simulink library "inp"  (R2021b)
settings: Solver=VariableStepAuto  StartTime=0.0  StopTime=10.0  RelTol=1e-3
undefined symbols (not defined in the file): C_TASK_5MS_S, FALSE, KINP_AcoreReadyToSlp_flg_ovrdflg, KINP_AcoreReadyToSlp_flg_ovrdval, KINP_AllowMovThd_OTA_enum_ovrdflg, KINP_AllowMovThd_OTA_enum_ovrdval, KINP_APSAngleTarget_Deg_ovrdflg, KINP_APSAngleTarget_Deg_ovrdval, KINP_APSDecReq_mps2_ovrdflg, KINP_APSDecReq_mps2_ovrdval, KINP_APSDecReqA_flg_ovrdflg, KINP_APSDecReqA_flg_ovrdval, KINP_APSDFLL_cm_ovrdflg, KINP_APSDFLL_cm_ovrdval, KINP_APSDFLR_cm_ovrdflg, KINP_APSDFLR_cm_ovrdval, KINP_APSDRLL_cm_ovrdflg, KINP_APSDRLL_cm_ovrdval, KINP_APSDRLR_cm_ovrdflg, KINP_APSDRLR_cm_ovrdval, KINP_APSExitCondition_enum_ovrdflg, KINP_APSExitCondition_enum_ovrdval, KINP_APSHWVer_enum_ovrdflg, KINP_APSHWVer_enum_ovrdval, KINP_APSProgressPCT_pct_ovrdflg, KINP_APSProgressPCT_pct_ovrdval, KINP_APSPwrReq_enum_ovrdflg, KINP_APSPwrReq_enum_ovrdval, KINP_APSReq_enum_ovrdflg, KINP_APSReq_enum_ovrdval, KINP_APSRQDisplay_enum_ovrdflg, KINP_APSRQDisplay_enum_ovrdval, KINP_APSRqEPASCtrl_flg_ovrdflg, KINP_APSRqEPASCtrl_flg_ovrdval, KINP_APSShiftPosnReq_enum_ovrdval, KINP_APSShiftPosnReq_enum_ovrflg, KINP_APSSpeedCMD_kph_ovrdval, KINP_APSSpeedCMD_kph_ovrflg, KINP_APSStaSystem_enum_ovrdflg, KINP_APSStaSystem_enum_ovrdval, KINP_APSSWVer_enum_ovrdflg, KINP_APSSWVer_enum_ovrdval, KINP_APSVMCReqA_flg_ovrdval, KINP_APSVMCReqA_flg_ovrflg, KINP_APSVRqEPASCtrl_flg_ovrdflg, KINP_APSVRqEPASCtrl_flg_ovrdval, KINP_AuxBattVolmV_mV_ovrdflg, KINP_AuxBattVolmV_mV_ovrdval, KINP_BTConnectSta_enum_ovrdflg, KINP_BTConnectSta_enum_ovrdval, KINP_CAASSta_enum_ovrdflg, KINP_CAASSta_enum_ovrdval, KINP_CAASVMCReqA_flg_ovrdval, KINP_CAASVMCReqA_flg_ovrflg, KINP_CAN1BusOff_flg_ovrdflg, KINP_CAN1BusOff_flg_ovrdval, KINP_CAN2BusOff_flg_ovrdflg, KINP_CAN2BusOff_flg_ovrdval, KINP_CAN3BusOff_flg_ovrdflg, KINP_CAN3BusOff_flg_ovrdval ... (+222)
libraries: FVT_lib x1035, hcu_lib x1
(part 2 of 33)

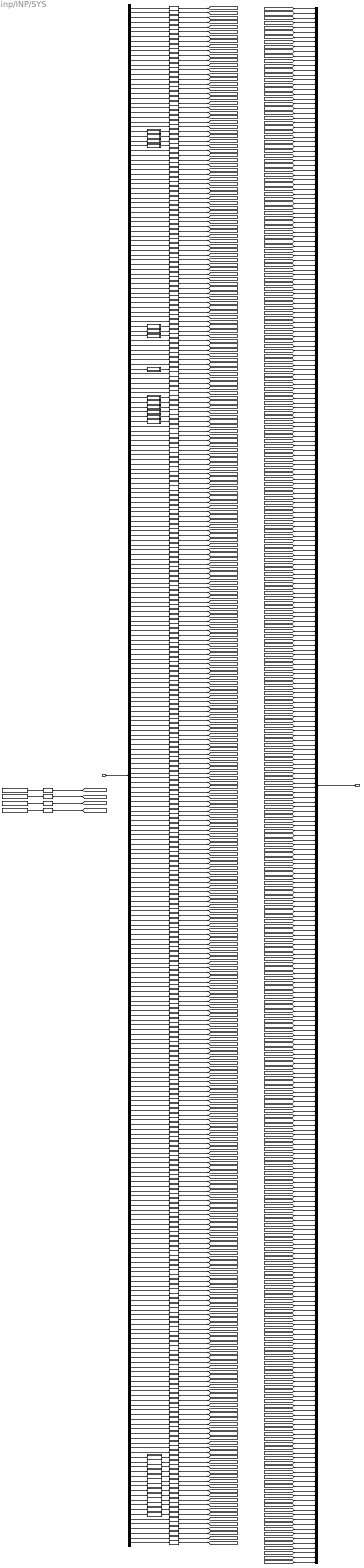
== system inp/INP/SYS ==
  BHAL_SYS_outputs : Inport  OutDataTypeStr=Bus: BHAL_SYS_outputs
  Bus Creator1 : BusCreator  Inputs=328  OutDataTypeStr=Bus: BINP_SYS_outputs  NonVirtualBus=on
  Bus Selector1 : BusSelector  OutputSignals=VHAL_CarMode1_cnt,VHAL_CarModel2_cnt,VHAL_CarModel3_cnt,VHAL_ECU1_cnt,VHAL_ECU2_cnt,VHAL_Major1_cnt,VHAL_Major2_cnt,VHAL_Minor1_cnt,VHAL_Minor2_cnt,VHAL_Patch1_cnt,VHAL_Patch2_cnt,VHAL_Country1_cnt,VHAL_Country2_cnt,VHAL_Variation_cnt,VHAL_Dash1_cnt,VHAL_Change1_cnt,VHAL_Change2_cnt,VHAL_Dash2_cnt,VHAL_SHA1_cnt,VHAL_SHA2_cnt,VHAL_SHA3_cnt,VHAL_SHA4_cnt,VHAL_SHA5_cnt,VHAL_SHA6_cnt,VHAL_SHA7_cnt,VHAL_SHA8_cnt,VHAL_AcoreReadyToSlp_flg,VHAL_PwrReq_OTA_enum,VHAL_AllowMovThd_OTA_enum,VHAL_EvccAplusPwrUpReq_flg,VHAL_DrivetrainSelect_enum,VHAL_ReadFlashCorrect_flg,VHAL_FlashAntitheft_enum,VHAL_RandomnumberY_raw1,VHAL_RandomnumberY_raw2,VHAL_RandomnumberY_raw3,VHAL_RandomnumberY_raw4,VHAL_RandomnumberY_raw5,VHAL_RandomnumberY_raw6,VHAL_RandomnumberY_raw7,VHAL_RandomnumberY_raw8,VHAL_FlashACModeSet123_enum,VHAL_FlashFace_enum,VHAL_FlashFoot_enum,VHAL_FlashFrost_enum,VHAL_FlashFaceM_enum,VHAL_FlashFootM_enum,VHAL_FlashCCUSyncSts_enum,VHAL_FlashACForceOFF_flg,VHAL_FlashsigRecircSt_enum,VHAL_FlashRecAutoFlg_enum,VHAL_FlashAirIntenZone1M_enum,VHAL_Flashfdefog_enum,VHAL_FlashsigSetTempZon1St_C,VHAL_FlashsigSetTempZon2StM_C,VHAL_FlashCountAlarm_enum,VHAL_FlashMFSWTri_flg,VHAL_FlashMirrorFlodPos_flg,VHAL_FlashFuelDoorPos_flg,VHAL_FlashLockSetting_enum,VHAL_FlashMFRDNBrightReq_pct,VHAL_FlashRoomLampMode_enum,VHAL_FlashWiperFixMode_flg,VHAL_FlashIVIPTGUSStaSW_enum,VHAL_AnyNMID_flg,VHAL_CurrentNmState_enum,VHAL_NvmProtectSta_flg,VHAL_AuxBattVolmV_mV,VHAL_Pedal1Ref5V_V,VHAL_Pedal2Ref5V_V,VHAL_EAPS1MINMem_pct,VHAL_EAPS2MINMem_pct,VHAL_FlashHoodSW_flg,VHAL_FlashTailgateSW_flg,VHAL_FlashCTDLockSW_flg,VHAL_FlashTailgateHDSW_flg,VHAL_NetworkReqCalled_flg,VHAL_PmicBootReason_enum,VHAL_WisrBootReason_raw32,VHAL_FlashAPMDoorControlSta_flg,VHAL_AcoreRebootCmd_flg,VHAL_DIDGetDynoMode_flg,VHAL_CAN1BusOff_flg,VHAL_CAN2BusOff_flg,VHAL_CAN3BusOff_flg,VHAL_CAN4BusOff_flg,VHAL_CAN5BusOff_flg,VHAL_CAN6BusOff_flg,VHAL_funAuto_flg,VHAL_DiagDRLOFF_flg,VHAL_DiagFMHT_s,VHAL_DiagFLTC_mA,VHAL_DiagFRTC_mA,VHAL_DiagRLTC_mA,VHAL_DiagRRTC_mA,VHAL_USSConfig_raw8,VHAL_TireSize_raw8,VHAL_APSFunConfig_raw8,VHAL_FlashfUnlockSingle_flg,VHAL_FlashRegenMode_enum,VHAL_FlashAmbFunEN_enum,VHAL_FlashAmbWelEN_enum,VHAL_FlashAmbDimEN_enum,VHAL_FlashAmbLinkDriSta_enum,VHAL_FlashAmbPwrWarnEN_enum,VHAL_FlashAmbODAEN_enum,VHAL_FlashAmbColorSta1_enum,VHAL_FlashAmbColorSta2_enum,VHAL_FlashAmbColorSta3_enum,VHAL_FlashAmbColorSta4_enum,VHAL_FlashAmbColorSta5_enum,VHAL_FlashAmbColorSta7_enum,VHAL_FlashAmbBrightnessSta1_enum,VHAL_FlashAmbBrightnessSta2_enum,VHAL_FlashAmbBrightnessSta3_enum,VHAL_FlashAmbBrightnessSta4_enum,VHAL_FlashAmbBrightnessSta5_enum,VHAL_FlashAmbBrightnessSta7_enum,VHAL_FlashTurnSwTSet123_enum,VHAL_FlashTurnSwTSet457_enum,VHAL_FlashAirIntZ3Sta_enum,VHAL_FlashREVentModeSta_enum,VHAL_FlashLEVentModeSta_enum,VHAL_FlashLEVentZSta_enum,VHAL_FlashCLEVentZSta_enum,VHAL_FlashREVentZSta_enum,VHAL_FlashCREVentZSta_enum,VHAL_FlashLVentEN_enum,VHAL_FlashLEVentYSta_enum,VHAL_FlashCLVentEN_enum,VHAL_FlashCLEVentYSta_enum,VHAL_FlashRVentEN_enum,VHAL_FlashREVentYSta_enum,VHAL_FlashCRVentEN_enum,VHAL_FlashCREVentYSta_enum,VHAL_FlashFGSAirIntSta_enum,VHAL_FlashFGSChSta_enum,VHAL_FlashFGSIONSWSta_enum,VHAL_FlashWalkOutLkEN_enum,VHAL_FlashWalkInUnLkEN_enum,VHAL_FlashFollowMeENFun_enum,VHAL_ResetPedalZeroPosReq_enum,VHAL_FlashPTGUserHeight1_cnt,VHAL_FlashPTGUserHeight2_cnt,VHAL_FlashPTGUserHeight3_cnt,VHAL_FlashPTGUserHeight4_cnt,VHAL_FlashPTGUserHeight5_cnt,VHAL_FlashPTGUserHeight7_cnt,VHAL_FlashPTGOpenHeight12_enum,VHAL_FlashPTGOpenHeight34_enum,VHAL_FlashPTGOpenHeight57_enum,VHAL_FlashACCLevelSta12_enum,VHAL_FlashACCLevelSta34_enum,VHAL_FlashACCLevelSta57_enum,VHAL_AutoWipHSpdEN_flg,VHAL_WipRLSCmdHoldEN_flg,VHAL_WipRLSCmdHoldTime_s,VHAL_WipRLSCmdCutEN_flg,VHAL_WipRLSCmdCutTime_s,VHAL_FlashAutoLock_enum,VHAL_FlashAutoUnlock_enum,VHAL_ECUGen1_cnt,VHAL_ECUGen2_cnt,VHAL_FlashMILDIST_km,VHAL_FlashWARMUPS_cnt,VHAL_FlashCLRDIST_km,VHAL_FlashMILTIME_min,VHAL_FlashCLRTIME_min,VHAL_FlashNUMPSATRIPSFLTMEMCLR_cnt,VHAL_FlashODOMETER_km,VHAL_FlashPSAR_sec,VHAL_FlashPSAL_sec,VHAL_FlashIPSAR_sec,VHAL_FlashIPSAL_sec,VHAL_FlashCPSAR_sec,VHAL_FlashCPSAL_sec,VHAL_FlashHVBNAH_Ahr,VHAL_FlashHVBNE_kWh,VHAL_FlashIGNCNTR_cnt,VHAL_FlashTNBCPSAR_Ahr,VHAL_FlashTNBCPSAL_Ahr,VHAL_FlashTNECPSAR_kWh,VHAL_FlashTNECPSAL_kWh,VHAL_FlashTEBPSAR_kWh,VHAL_FlashTEBPSAL_kWh,VHAL_FlashTGEOVCR_kWh,VHAL_FlashTGEOVCL_kWh,VHAL_FlashGECHGOVCDCR_kWh,VHAL_FlashGECHGOVCDCL_kWh,VHAL_FlashGECHGOVCACR_kWh,VHAL_FlashGECHGOVCACL_kWh,VHAL_FlashRESSV2XENNONPSAR_kWh,VHAL_FlashRESSV2XENNONPSAL_kWh,VHAL_FlashPKERNumerator_kphsqr,VHAL_FlashPKELNumerator_kphsqr,VHAL_FlashResetCDEODTR_km,VHAL_FlashAvgBattTempPSAR_C,VHAL_FlashAvgBattTempPSAL_C,VHAL_FlashAvgBattTempOVCR_C,VHAL_FlashAvgBattTempOVCL_C,VHAL_FlashAvgBattTempOFFR_C,VHAL_FlashAvgBattTempOFFL_C,VHAL_FlashQTYPSATRIPSR_cnt,VHAL_FlashQTYPSATRIPSL_cnt,VHAL_FlashRESSCNTDODRNGR_cnt,VHAL_FlashRESSCNTDODRNGL_cnt,VHAL_FlashETMATOER_kWh,VHAL_FlashETMATOEL_kWh,VHAL_FlashETMBTOER_kWh,VHAL_FlashETMBTOEL_kWh,VHAL_FlashRESSTIMESOCPSARNGR_s,VHAL_FlashRESSTIMESOCPSARNGL_s,VHAL_FlashRESSTIMESOCCHGRNGR_s,VHAL_FlashRESSTIMESOCCHGRNGL_s,VHAL_FlashRESSTIMESOCOFFRNGR_s,VHAL_FlashRESSTIMESOCOFFRNGL_s,VHAL_FlashMAXBATTEMPL_C,VHAL_FlashMINBATTEMPL_C,VHAL_FlashAVGBATTEMPL_sec,VHAL_FlashAVGBATTEMPL_C,VHAL_FlashBattTempPSAR_sec,VHAL_FlashBattTempPSAL_sec,VHAL_FlashOVCR_sec,VHAL_FlashOVCL_sec,VHAL_FlashOFFR_sec,VHAL_FlashOFFL_sec,VHAL_VinCode_cnt,VHAL_FlashHMIKey1Func_enum,VHAL_FlashHMIKey2Func_enum,VHAL_FlashHMIKey3Func_enum,VHAL_FlashHMIKey4Func_enum,VHAL_FlashHMIKey5Func_enum,VHAL_FlashHMIKey6Func_enum,VHAL_FlashHMIKey7Func_enum,VHAL_FlashHMIKey8Func_enum,VHAL_FlashAutoWipHSpdEN_flg,VHAL_PmicBootPath_raw32,VHAL_FlashTPMModelVersion_raw,VHAL_FlashTPMModelVersionChkSum_raw,VHAL_FlashDIDModelVersion_raw,VHAL_FlashDIDModelVersionChkSum_raw,VHAL_FlashAirIntenZone1MSet2_enum,VHAL_FlashAirIntenZone1MSet3_enum,VHAL_FlashAirIntenZone1MSet4_enum,VHAL_FlashAirIntenZone1MSet5_enum,VHAL_FlashAirIntenZone1MSet7_enum,VHAL_FlashAirIntenZone3MSet2_enum,VHAL_FlashAirIntenZone3MSet3_enum,VHAL_FlashAirIntenZone3MSet4_enum,VHAL_FlashAirIntenZone3MSet5_enum,VHAL_FlashAirIntenZone3MSet7_enum,VHAL_FlashFGSChStaSet457_enum,VHAL_FlashFGSAirIntStaSet457_enum,VHAL_FlashLEVentModeStaSet457_enum,VHAL_FlashREVentModeStaSet457_enum,VHAL_FlashLEVentZStaSet2_enum,VHAL_FlashLEVentZStaSet3_enum,VHAL_FlashLEVentZStaSet4_enum,VHAL_FlashLEVentZStaSet5_enum,VHAL_FlashLEVentZStaSet7_enum,VHAL_FlashCLEVentZStaSet2_enum,VHAL_FlashCLEVentZStaSet3_enum,VHAL_FlashCLEVentZStaSet4_enum,VHAL_FlashCLEVentZStaSet5_enum,VHAL_FlashCLEVentZStaSet7_enum,VHAL_FlashREVentZStaSet2_enum,VHAL_FlashREVentZStaSet3_enum,VHAL_FlashREVentZStaSet4_enum,VHAL_FlashREVentZStaSet5_enum,VHAL_FlashREVentZStaSet7_enum,VHAL_FlashCREVentZStaSet2_enum,VHAL_FlashCREVentZStaSet3_enum,VHAL_FlashCREVentZStaSet4_enum,VHAL_FlashCREVentZStaSet5_enum,VHAL_FlashCREVentZStaSet7_enum,VHAL_FlashLEVentYStaSet2_enum,VHAL_FlashLEVentYStaSet3_enum,VHAL_FlashLEVentYStaSet4_enum,VHAL_FlashLEVentYStaSet5_enum,VHAL_FlashLEVentYStaSet7_enum,VHAL_FlashCLEVentYStaSet2_enum,VHAL_FlashCLEVentYStaSet3_enum,VHAL_FlashCLEVentYStaSet4_enum,VHAL_FlashCLEVentYStaSet5_enum,VHAL_FlashCLEVentYStaSet7_enum,VHAL_FlashREVentYStaSet2_enum,VHAL_FlashREVentYStaSet3_enum,VHAL_FlashREVentYStaSet4_enum,VHAL_FlashREVentYStaSet5_enum,VHAL_FlashREVentYStaSet7_enum,VHAL_FlashCREVentYStaSet2_enum,VHAL_FlashCREVentYStaSet3_enum,VHAL_FlashCREVentYStaSet4_enum,VHAL_FlashCREVentYStaSet5_enum,VHAL_FlashCREVentYStaSet7_enum,VHAL_FlashACModeSet457_enum,VHAL_FlashSettempZon1Set2_enum,VHAL_FlashSettempZon1Set3_enum,VHAL_FlashSettempZon1Set4_enum,VHAL_FlashSettempZon1Set5_enum,VHAL_FlashSettempZon1Set7_enum,VHAL_FlashJugKeepUnLZone_flg,VHAL_DrivingMode_cnt,VHAL_ModelYear_cnt,VHAL_FlashCLWinLockDrSta_enum,VHAL_CbnPreACEnaReq_enum,VHAL_PowerOffTSet_cnt,VHAL_ReOutsideMirror_enum,VHAL_ReDoorLock_enum,VHAL_RePwrReqTbox_enum,VHAL_ReRadio_flg,VHAL_RemoteACTemp_C,VHAL_RemoteAutoReq_flg,VHAL_TBOXRemotePW_enum,VHAL_FDCConnDrvWdwCtrlCmd_pct,VHAL_FDCConnPasWdwCtrlCmd_pct,VHAL_FDCConnRLDWdwCtrlCmd_pct,VHAL_FDCConnRRDWdwCtrlCmd_pct,VHAL_CAN1BusError_flg,VHAL_CAN2BusError_flg,VHAL_CAN3BusError_flg,VHAL_CAN4BusError_flg,VHAL_CAN5BusError_flg,VHAL_CAN6BusError_flg
  Constant : Constant  Value=KINP_NewNMSpec_flg
  Constant1 : Constant  Value=KINP_VehicleType_enum
  Constant2 : Constant  Value=KINP_SWCType_enum
  Constant3 : Constant  Value=KINP_SOCDisUsed_flg
  Data Type Conversion{,4,6,12..16,19..27,36,54,57..58,78,81,89,102,112,137..139,147,238,305,314,316,322..327} (40 alike) : DataTypeConversion  OutDataTypeStr=boolean
  Data Type Conversion{1..3,5,17,33..35,37..53,55..56,59..77,79..80,82..88,90..101,103..111,113..122,129..136,140..141,145..146,148,192..209,229..237,240..243,245..304,306..309,311,313,317..321} (201 alike) : DataTypeConversion  OutDataTypeStr=uint8
  Data Type Conversion{8..11,28..32,149..150,154,161..162,164..177,180..186,191,210..212,219..221,310,315} (44 alike) : DataTypeConversion  OutDataTypeStr=single
  Data Type Conversion{7,123..128,151..153,163,189..190,312} (14 alike) : DataTypeConversion  OutDataTypeStr=uint16
  Data Type Conversion{142..144,244} (4 alike) : DataTypeConversion
  Data Type Conversion{18,155..160,178..179,187..188,213..218,222..228,239} (25 alike) : DataTypeConversion  OutDataTypeStr=uint32
  Subsystem : Subsystem
  Subsystem1 : Subsystem
  Subsystem10 : Subsystem
  Subsystem11 : Subsystem
  Subsystem12 : Subsystem
  Subsystem13 : Subsystem
  Subsystem14 : Subsystem
  Subsystem15 : Subsystem
  Subsystem16 : Subsystem
  Subsystem17 : Subsystem
  Subsystem18 : Subsystem
  Subsystem19 : Subsystem
  Subsystem2 : Subsystem
  Subsystem20 : Subsystem
  Subsystem21 : Subsystem
  Subsystem22 : Subsystem
  Subsystem23 : Subsystem
  Subsystem24 : Subsystem
  Subsystem25 : Subsystem
  Subsystem26 : Subsystem
  Subsystem3 : Subsystem
  Subsystem4 : Subsystem
  Subsystem5 : Subsystem
  Subsystem6 : Subsystem
  Subsystem7 : Subsystem
  Subsystem8 : Subsystem
  Subsystem9 : Subsystem
  BINP_SYS_outputs : Outport  OutDataTypeStr=Bus: BINP_SYS_outputs
  wires:
  [VINP_Country2_cnt] -> Bus Creator1/13
  [VINP_FlashAirIntenZone1M_enum] -> Bus Creator1/52
  [VINP_FlashFrost_enum] -> Bus Creator1/45
  Bus Selector1/43 -> Data Type Conversion96/1  "<VHAL_FlashFace_enum>"
  [VINP_FlashCCUSyncSts_enum] -> Bus Creator1/48
  [VINP_EvccAplusPwrUpReq_flg] -> Bus Creator1/30
  Data Type Conversion110/1 -> [VINP_Minor2_cnt]  "VINP_Minor2_cnt"
  Bus Selector1/53 -> Data Type Conversion107/1  "<VHAL_Flashfdefog_enum>"
  [VINP_FlashRecAutoFlg_enum] -> Bus Creator1/51
  Bus Selector1/16 -> Data Type Conversion66/1  "<VHAL_Change1_cnt>"
  [VINP_RandomnumberY_raw1] -> Bus Creator1/34
  Data Type Conversion97/1 -> [VINP_FlashFoot_enum]  "VINP_FlashFoot_enum"
  Bus Selector1/44 -> Data Type Conversion97/1  "<VHAL_FlashFoot_enum>"
  [VINP_FlashFoot_enum] -> Bus Creator1/44
  [VINP_FlashFootM_enum] -> Bus Creator1/47
  Data Type Conversion72/1 -> [VINP_SHA3_cnt]  "VINP_SHA3_cnt"
  [VINP_FlashsigRecircSt_enum] -> Bus Creator1/50
  Data Type Conversion60/1 -> [VINP_CarModel2_cnt]  "VINP_CarModel2_cnt"
  Data Type Conversion100/1 -> [VINP_FlashFootM_enum]  "VINP_FlashFootM_enum"
  Bus Selector1/3 -> Data Type Conversion71/1  "<VHAL_CarModel3_cnt>"
  Data Type Conversion104/1 -> [VINP_Major1_cnt]  "VINP_Major1_cnt"
  [VINP_FlashFaceM_enum] -> Bus Creator1/46
  [VINP_Dash1_cnt] -> Bus Creator1/15
  Bus Selector1/45 -> Data Type Conversion98/1  "<VHAL_FlashFrost_enum>"
  [VINP_FlashACModeMem_enum] -> Bus Creator1/42
  Data Type Conversion108/1 -> [VINP_Major2_cnt]  "VINP_Major2_cnt"
  [VINP_FlashFace_enum] -> Bus Creator1/43
  Bus Selector1/8 -> Data Type Conversion109/1  "<VHAL_Minor1_cnt>"
  [VINP_CarModel1_cnt] -> Bus Creator1/1
  Data Type Conversion82/1 -> [VINP_ECU1_cnt]  "VINP_ECU1_cnt"
  Bus Selector1/47 -> Data Type Conversion100/1  "<VHAL_FlashFootM_enum>"
  Data Type Conversion73/1 -> [VINP_SHA4_cnt]  "VINP_SHA4_cnt"
  Bus Selector1/34 -> Data Type Conversion85/1  "<VHAL_RandomnumberY_raw1>"
  Data Type Conversion84/1 -> [VINP_DrivetrainSelect_enum]  "VINP_DrivetrainSelect_enum"
  Bus Selector1/30 -> Subsystem6/1(In1)  "<VHAL_EvccAplusPwrUpReq_flg>"
  Data Type Conversion101/1 -> [VINP_FlashCCUSyncSts_enum]  "VINP_FlashCCUSyncSts_enum"
  [VINP_DrivetrainSelect_enum] -> Bus Creator1/31
  Data Type Conversion80/1 -> [VINP_AllowMovThd_OTA_enum]  "VINP_AllowMovThd_OTA_enum"
  Bus Selector1/49 -> Data Type Conversion102/1  "<VHAL_FlashACForceOFF_flg>"
  Bus Selector1/38 -> Data Type Conversion90/1  "<VHAL_RandomnumberY_raw5>"
  Bus Selector1/10 -> Data Type Conversion111/1  "<VHAL_Patch1_cnt>"
  Data Type Conversion88/1 -> [VINP_RandomnumberY_raw4]  "VINP_RandomnumberY_raw4"
  [VINP_Flashfdefog_enum] -> Bus Creator1/53
  Bus Selector1/42 -> Data Type Conversion95/1  "<VHAL_FlashACModeSet123_enum>"
  Bus Selector1/37 -> Data Type Conversion88/1  "<VHAL_RandomnumberY_raw4>"
  Bus Selector1/36 -> Data Type Conversion87/1  "<VHAL_RandomnumberY_raw3>"
  Bus Selector1/48 -> Data Type Conversion101/1  "<VHAL_FlashCCUSyncSts_enum>"
  Data Type Conversion102/1 -> [VINP_FlashACForceOFF_flg]  "VINP_FlashACForceOFF_flg"
  [VINP_Change2_cnt] -> Bus Creator1/17
  Bus Selector1/29 -> Subsystem5/1(In1)  "<VHAL_AllowMovThd_OTA_enum>"
  Data Type Conversion63/1 -> [VINP_Country2_cnt]  "VINP_Country2_cnt"
  Data Type Conversion107/1 -> [VINP_Flashfdefog_enum]  "VINP_Flashfdefog_enum"
  Data Type Conversion96/1 -> [VINP_FlashFace_enum]  "VINP_FlashFace_enum"
  [VINP_RandomnumberY_raw2] -> Bus Creator1/35
  [VINP_RandomnumberY_raw6] -> Bus Creator1/39
  [VINP_RandomnumberY_raw4] -> Bus Creator1/37
  [VINP_ECU1_cnt] -> Bus Creator1/4
  Bus Selector1/2 -> Data Type Conversion60/1  "<VHAL_CarModel2_cnt>"
  Data Type Conversion105/1 -> [VINP_FlashRecAutoFlg_enum]  "VINP_FlashRecAutoFlg_enum"
  Data Type Conversion103/1 -> [VINP_FlashsigRecircSt_enum]  "VINP_FlashsigRecircSt_enum"
  Bus Selector1/22 -> Data Type Conversion73/1  "<VHAL_SHA4_cnt>"
  Bus Selector1/46 -> Data Type Conversion99/1  "<VHAL_FlashFaceM_enum>"
  Bus Selector1/50 -> Data Type Conversion103/1  "<VHAL_FlashsigRecircSt_enum>"
  Data Type Conversion98/1 -> [VINP_FlashFrost_enum]  "VINP_FlashFrost_enum"
  [VINP_RandomnumberY_raw5] -> Bus Creator1/38
  [VINP_SHA3_cnt] -> Bus Creator1/21
  Bus Selector1/40 -> Data Type Conversion92/1  "<VHAL_RandomnumberY_raw7>"
  Data Type Conversion86/1 -> [VINP_RandomnumberY_raw2]  "VINP_RandomnumberY_raw2"
  Data Type Conversion111/1 -> [VINP_Patch1_cnt]  "VINP_Patch1_cnt"
  Bus Selector1/35 -> Data Type Conversion86/1  "<VHAL_RandomnumberY_raw2>"
  [VINP_SHA6_cnt] -> Bus Creator1/24
  [VINP_Major1_cnt] -> Bus Creator1/6
  [VINP_RandomnumberY_raw7] -> Bus Creator1/40
  [VINP_RandomnumberY_raw8] -> Bus Creator1/41
  Bus Selector1/15 -> Data Type Conversion65/1  "<VHAL_Dash1_cnt>"
  Data Type Conversion92/1 -> [VINP_RandomnumberY_raw7]  "VINP_RandomnumberY_raw7"
  Data Type Conversion99/1 -> [VINP_FlashFaceM_enum]  "VINP_FlashFaceM_enum"
  Data Type Conversion85/1 -> [VINP_RandomnumberY_raw1]  "VINP_RandomnumberY_raw1"
  Bus Selector1/52 -> Data Type Conversion106/1  "<VHAL_FlashAirIntenZone1M_enum>"
  Data Type Conversion90/1 -> [VINP_RandomnumberY_raw5]  "VINP_RandomnumberY_raw5"
  Data Type Conversion91/1 -> [VINP_RandomnumberY_raw6]  "VINP_RandomnumberY_raw6"
  Data Type Conversion65/1 -> [VINP_Dash1_cnt]  "VINP_Dash1_cnt"
  [VINP_FlashAntitheft_enum] -> Bus Creator1/33
  Data Type Conversion87/1 -> [VINP_RandomnumberY_raw3]  "VINP_RandomnumberY_raw3"
  Bus Selector1/39 -> Data Type Conversion91/1  "<VHAL_RandomnumberY_raw6>"
  [VINP_Dash2_cnt] -> Bus Creator1/18
  Bus Selector1/19 -> Data Type Conversion69/1  "<VHAL_SHA1_cnt>"
  Bus Selector1/41 -> Data Type Conversion94/1  "<VHAL_RandomnumberY_raw8>"
  Data Type Conversion71/1 -> [VINP_CarModel3_cnt]  "VINP_CarModel3_cnt"
  [VINP_SHA4_cnt] -> Bus Creator1/22
  Data Type Conversion76/1 -> [VINP_SHA7_cnt]  "VINP_SHA7_cnt"
  [VINP_AllowMovThd_OTA_enum] -> Bus Creator1/29
  [VINP_ReadFlashCorrect_flg] -> Bus Creator1/32
  Data Type Conversion78/1 -> [VINP_AcoreReadyToSlp_flg]  "VINP_AcoreReadyToSlp_flg"
  Data Type Conversion94/1 -> [VINP_RandomnumberY_raw8]  "VINP_RandomnumberY_raw8"
  Data Type Conversion67/1 -> [VINP_Change2_cnt]  "VINP_Change2_cnt"
  [VINP_CarModel3_cnt] -> Bus Creator1/3
  [VINP_Variation_cnt] -> Bus Creator1/14
  [VINP_SHA2_cnt] -> Bus Creator1/20
  [VINP_FlashACForceOFF_flg] -> Bus Creator1/49
  Bus Selector1/12 -> Data Type Conversion62/1  "<VHAL_Country1_cnt>"
  Bus Selector1/51 -> Data Type Conversion105/1  "<VHAL_FlashRecAutoFlg_enum>"
  Data Type Conversion69/1 -> [VINP_SHA1_cnt]  "VINP_SHA1_cnt"
  [VINP_AcoreReadyToSlp_flg] -> Bus Creator1/27
  [VINP_PwrReq_OTA_enum] -> Bus Creator1/28
  Subsystem4/1(Out1) -> Data Type Conversion79/1
  [VINP_SHA5_cnt] -> Bus Creator1/23
  [VINP_Patch2_cnt] -> Bus Creator1/11
  [VINP_Patch1_cnt] -> Bus Creator1/10
  Data Type Conversion68/1 -> [VINP_Dash2_cnt]  "VINP_Dash2_cnt"
  Subsystem6/1(Out1) -> Data Type Conversion89/1
  Bus Selector1/33 -> Data Type Conversion83/1  "<VHAL_FlashAntitheft_enum>"
  [VINP_Minor2_cnt] -> Bus Creator1/9
  [VINP_SHA7_cnt] -> Bus Creator1/25
  [VINP_Minor1_cnt] -> Bus Creator1/8
  Data Type Conversion95/1 -> [VINP_FlashACModeMem_enum]  "VINP_FlashACModeMem_enum"
  [VINP_CarModel2_cnt] -> Bus Creator1/2
  Data Type Conversion77/1 -> [VINP_SHA8_cnt]  "VINP_SHA8_cnt"
  Data Type Conversion106/1 -> [VINP_FlashAirIntenZone1M_enum]  "VINP_FlashAirIntenZone1M_enum"
  Data Type Conversion66/1 -> [VINP_Change1_cnt]  "VINP_Change1_cnt"
  [VINP_SHA1_cnt] -> Bus Creator1/19
  Data Type Conversion81/1 -> [VINP_ReadFlashCorrect_flg]  "VINP_ReadFlashCorrect_flg"
  [VINP_Country1_cnt] -> Bus Creator1/12
  Bus Selector1/17 -> Data Type Conversion67/1  "<VHAL_Change2_cnt>"
  Data Type Conversion83/1 -> [VINP_FlashAntitheft_enum]  "VINP_FlashAntitheft_enum"
  Data Type Conversion75/1 -> [VINP_SHA6_cnt]  "VINP_SHA6_cnt"
  Data Type Conversion74/1 -> [VINP_SHA5_cnt]  "VINP_SHA5_cnt"
  Data Type Conversion93/1 -> [VINP_ECU2_cnt]  "VINP_ECU2_cnt"
  [VINP_RandomnumberY_raw3] -> Bus Creator1/36
  Data Type Conversion70/1 -> [VINP_SHA2_cnt]  "VINP_SHA2_cnt"
  Bus Selector1/21 -> Data Type Conversion72/1  "<VHAL_SHA3_cnt>"
  Data Type Conversion62/1 -> [VINP_Country1_cnt]  "VINP_Country1_cnt"
  [VINP_ECU2_cnt] -> Bus Creator1/5
  Bus Selector1/31 -> Data Type Conversion84/1  "<VHAL_DrivetrainSelect_enum>"
  Data Type Conversion64/1 -> [VINP_Variation_cnt]  "VINP_Variation_cnt"
  Data Type Conversion61/1 -> [VINP_Patch2_cnt]  "VINP_Patch2_cnt"
  Bus Selector1/18 -> Data Type Conversion68/1  "<VHAL_Dash2_cnt>"
  Bus Selector1/28 -> Subsystem4/1(In1)  "<VHAL_PwrReq_OTA_enum>"
  Bus Selector1/24 -> Data Type Conversion75/1  "<VHAL_SHA6_cnt>"
  Bus Selector1/27 -> Subsystem7/1(In1)  "<VHAL_AcoreReadyToSlp_flg>"
  [VINP_SHA8_cnt] -> Bus Creator1/26
  Bus Selector1/20 -> Data Type Conversion70/1  "<VHAL_SHA2_cnt>"
  Subsystem5/1(Out1) -> Data Type Conversion80/1
  Bus Selector1/25 -> Data Type Conversion76/1  "<VHAL_SHA7_cnt>"
  [VINP_Major2_cnt] -> Bus Creator1/7
  Bus Selector1/32 -> Data Type Conversion81/1  "<VHAL_ReadFlashCorrect_flg>"
  Data Type Conversion59/1 -> [VINP_CarModel1_cnt]  "VINP_CarModel1_cnt"
  Bus Selector1/23 -> Data Type Conversion74/1  "<VHAL_SHA5_cnt>"
  Bus Selector1/14 -> Data Type Conversion64/1  "<VHAL_Variation_cnt>"
  [VINP_Change1_cnt] -> Bus Creator1/16
  Subsystem7/1(Out1) -> Data Type Conversion78/1
  Bus Selector1/13 -> Data Type Conversion63/1  "<VHAL_Country2_cnt>"
  Bus Selector1/4 -> Data Type Conversion82/1  "<VHAL_ECU1_cnt>"
  Data Type Conversion79/1 -> [VINP_PwrReq_OTA_enum]  "VINP_PwrReq_OTA_enum"
  Bus Selector1/7 -> Data Type Conversion108/1  "<VHAL_Major2_cnt>"
  Bus Selector1/9 -> Data Type Conversion110/1  "<VHAL_Minor2_cnt>"
  Bus Selector1/5 -> Data Type Conversion93/1  "<VHAL_ECU2_cnt>"
  Data Type Conversion89/1 -> [VINP_EvccAplusPwrUpReq_flg]  "VINP_EvccAplusPwrUpReq_flg"
  Bus Selector1/1 -> Data Type Conversion59/1  "<VHAL_CarMode1_cnt>"
  Bus Selector1/6 -> Data Type Conversion104/1  "<VHAL_Major1_cnt>"
  Data Type Conversion109/1 -> [VINP_Minor1_cnt]  "VINP_Minor1_cnt"
  BHAL_SYS_outputs/1 -> Bus Selector1/1
  Bus Creator1/1 -> BINP_SYS_outputs/1
  Bus Selector1/11 -> Data Type Conversion61/1  "<VHAL_Patch2_cnt>"
  Bus Selector1/26 -> Data Type Conversion77/1  "<VHAL_SHA8_cnt>"
  Data Type Conversion112/1 -> [VINP_AnyNMID_flg]  "VINP_AnyNMID_flg"
  Data Type Conversion113/1 -> [VINP_CurrentNmState_enum]  "VINP_CurrentNmState_enum"
  Bus Selector1/65 -> Data Type Conversion112/1  "<VHAL_AnyNMID_flg>"
  Bus Selector1/66 -> Data Type Conversion113/1  "<VHAL_CurrentNmState_enum>"
  Data Type Conversion56/1 -> [VINP_FlashCountAlarm_enum]  "VINP_FlashCountAlarm_enum"
  Data Type Conversion4/1 -> [VINP_FlashWiperFixMode_flg]  "VINP_FlashWiperFixMode_flg"
  Data Type Conversion3/1 -> [VINP_FlashRoomLampMode_enum]  "VINP_FlashRoomLampMode_enum"
  Data Type Conversion57/1 -> [VINP_FlashMirrorFlodPos_flg]  "VINP_FlashMirrorFlodPos_flg"
  Data Type Conversion55/1 -> [VINP_FlashsigSetTempZon2StM_C]  "VINP_FlashsigSetTempZon2StM_C"
  Data Type Conversion54/1 -> [VINP_FlashMFSWTri_flg]  "VINP_FlashMFSWTri_flg"
  Data Type Conversion58/1 -> [VINP_FlashFuelDoorPos_flg]  "VINP_FlashFuelDoorPos_flg"
  Data Type Conversion53/1 -> [VINP_FlashsigSetTempZon1St_C]  "VINP_FlashsigSetTempZon1St_C"
  Data Type Conversion5/1 -> [VINP_FlashIVIPTGUSStaSW_enum]  "VINP_FlashIVIPTGUSStaSW_enum"
  Data Type Conversion2/1 -> [VINP_FlashMFRDNBrightReq_pct]  "VINP_FlashMFRDNBrightReq_pct"
  Data Type Conversion1/1 -> [VINP_FlashLockSetting_enum]  "VINP_FlashLockSetting_enum"
  Bus Selector1/54 -> Data Type Conversion53/1  "<VHAL_FlashsigSetTempZon1St_C>"
  Bus Selector1/55 -> Data Type Conversion55/1  "<VHAL_FlashsigSetTempZon2StM_C>"
  Bus Selector1/56 -> Data Type Conversion56/1  "<VHAL_FlashCountAlarm_enum>"
  Bus Selector1/57 -> Data Type Conversion54/1  "<VHAL_FlashMFSWTri_flg>"
  Bus Selector1/58 -> Data Type Conversion57/1  "<VHAL_FlashMirrorFlodPos_flg>"
  Bus Selector1/59 -> Data Type Conversion58/1  "<VHAL_FlashFuelDoorPos_flg>"
  Bus Selector1/60 -> Data Type Conversion1/1  "<VHAL_FlashLockSetting_enum>"
  Bus Selector1/61 -> Data Type Conversion2/1  "<VHAL_FlashMFRDNBrightReq_pct>"
  Bus Selector1/62 -> Data Type Conversion3/1  "<VHAL_FlashRoomLampMode_enum>"
  Bus Selector1/63 -> Data Type Conversion4/1  "<VHAL_FlashWiperFixMode_flg>"
  Bus Selector1/64 -> Data Type Conversion5/1  "<VHAL_FlashIVIPTGUSStaSW_enum>"
  [VINP_FlashsigSetTempZon1St_C] -> Bus Creator1/54
  [VINP_FlashsigSetTempZon2StM_C] -> Bus Creator1/55
  [VINP_FlashCountAlarm_enum] -> Bus Creator1/56
  [VINP_FlashMFSWTri_flg] -> Bus Creator1/57
  [VINP_FlashMirrorFlodPos_flg] -> Bus Creator1/58
  [VINP_FlashFuelDoorPos_flg] -> Bus Creator1/59
  [VINP_FlashLockSetting_enum] -> Bus Creator1/60
  [VINP_FlashMFRDNBrightReq_pct] -> Bus Creator1/61
  [VINP_FlashRoomLampMode_enum] -> Bus Creator1/62
  [VINP_FlashWiperFixMode_flg] -> Bus Creator1/63
  [VINP_FlashIVIPTGUSStaSW_enum] -> Bus Creator1/64
  [VINP_AnyNMID_flg] -> Bus Creator1/65
  [VINP_CurrentNmState_enum] -> Bus Creator1/66
  Bus Selector1/67 -> Data Type Conversion6/1  "<VHAL_NvmProtectSta_flg>"
  Data Type Conversion6/1 -> [VINP_NvmProtectSta_flg]  "VINP_NvmProtectSta_flg"
  [VINP_NvmProtectSta_flg] -> Bus Creator1/67
  Bus Selector1/68 -> Subsystem/1(In1)  "<VHAL_AuxBattVolmV_mV>"
  Bus Selector1/69 -> Subsystem2/1(In1)  "<VHAL_Pedal1Ref5V_V>"
  Bus Selector1/70 -> Subsystem3/1(In1)  "<VHAL_Pedal2Ref5V_V>"
  Bus Selector1/71 -> Data Type Conversion10/1  "<VHAL_EAPS1MINMem_pct>"
  Bus Selector1/72 -> Data Type Conversion11/1  "<VHAL_EAPS2MINMem_pct>"
  Data Type Conversion7/1 -> [VINP_AuxBattVolmV_mV]  "VINP_AuxBattVolmV_mV"
  Data Type Conversion8/1 -> [VINP_Pedal1Ref5V_V]  "VINP_Pedal1Ref5V_V"
  Data Type Conversion9/1 -> [VINP_Pedal2Ref5V_V]  "VINP_Pedal2Ref5V_V"
  Data Type Conversion10/1 -> [VINP_EAPS1MINMem_pct]  "VINP_EAPS1MINMem_pct"
  Data Type Conversion11/1 -> [VINP_EAPS2MINMem_pct]  "VINP_EAPS2MINMem_pct"
  [VINP_AuxBattVolmV_mV] -> Bus Creator1/68
  [VINP_Pedal1Ref5V_V] -> Bus Creator1/69
  [VINP_Pedal2Ref5V_V] -> Bus Creator1/70
  [VINP_EAPS1MINMem_pct] -> Bus Creator1/71
  [VINP_EAPS2MINMem_pct] -> Bus Creator1/72
  Bus Selector1/73 -> Data Type Conversion12/1  "<VHAL_FlashHoodSW_flg>"
  Bus Selector1/74 -> Data Type Conversion13/1  "<VHAL_FlashTailgateSW_flg>"
  Bus Selector1/75 -> Data Type Conversion14/1  "<VHAL_FlashCTDLockSW_flg>"
  Bus Selector1/76 -> Data Type Conversion15/1  "<VHAL_FlashTailgateHDSW_flg>"
  Data Type Conversion12/1 -> [VINP_FlashHoodSW_flg]  "VINP_FlashHoodSW_flg"
  Data Type Conversion13/1 -> [VINP_FlashTailgateSW_flg]  "VINP_FlashTailgateSW_flg"
  Data Type Conversion14/1 -> [VINP_FlashCTDLockSW_flg]  "VINP_FlashCTDLockSW_flg"
  Data Type Conversion15/1 -> [VINP_FlashTailgateHDSW_flg]  "VINP_FlashTailgateHDSW_flg"
  [VINP_FlashHoodSW_flg] -> Bus Creator1/73
  [VINP_FlashTailgateSW_flg] -> Bus Creator1/74
  [VINP_FlashCTDLockSW_flg] -> Bus Creator1/75
  [VINP_FlashTailgateHDSW_flg] -> Bus Creator1/76
  Subsystem/1(Out1) -> Data Type Conversion7/1
  Bus Selector1/77 -> Subsystem1/1(In1)  "<VHAL_NetworkReqCalled_flg>"
  Data Type Conversion16/1 -> [VINP_NetworkReqCalled_flg]  "VINP_NetworkReqCalled_flg"
  Subsystem1/1(Out1) -> Data Type Conversion16/1
  [VINP_NetworkReqCalled_flg] -> Bus Creator1/77
  Bus Selector1/78 -> Data Type Conversion17/1  "<VHAL_PmicBootReason_enum>"
  Bus Selector1/79 -> Data Type Conversion18/1  "<VHAL_WisrBootReason_raw32>"
  Bus Selector1/80 -> Data Type Conversion19/1  "<VHAL_FlashAPMDoorControlSta_flg>"
  Data Type Conversion17/1 -> [VINP_PmicBootReason_enum]  "VINP_PmicBootReason_enum"
  Data Type Conversion18/1 -> [VINP_WisrBootReason_raw32]  "VINP_WisrBootReason_raw32"
  Data Type Conversion19/1 -> [VINP_FlashAPMDoorControlSta_flg]  "VINP_FlashAPMDoorControlSta_flg"
  [VINP_PmicBootReason_enum] -> Bus Creator1/78
  [VINP_WisrBootReason_raw32] -> Bus Creator1/79
  [VINP_FlashAPMDoorControlSta_flg] -> Bus Creator1/80
  Subsystem2/1(Out1) -> Data Type Conversion8/1
  Subsystem3/1(Out1) -> Data Type Conversion9/1
  Bus Selector1/81 -> Data Type Conversion20/1  "<VHAL_AcoreRebootCmd_flg>"
  Data Type Conversion20/1 -> [VINP_AcoreRebootCmd_flg]  "VINP_AcoreRebootCmd_flg"
  [VINP_AcoreRebootCmd_flg] -> Bus Creator1/81
  Bus Selector1/82 -> Data Type Conversion21/1  "<VHAL_DIDGetDynoMode_flg>"
  Data Type Conversion21/1 -> [VINP_DIDGetDynoMode_flg]  "VINP_DIDGetDynoMode_flg"
  [VINP_DIDGetDynoMode_flg] -> Bus Creator1/82
  Bus Selector1/83 -> Subsystem8/1(In1)  "<VHAL_CAN1BusOff_flg>"
  Bus Selector1/84 -> Subsystem9/1(In1)  "<VHAL_CAN2BusOff_flg>"
  Bus Selector1/85 -> Subsystem10/1(In1)  "<VHAL_CAN3BusOff_flg>"
  Bus Selector1/86 -> Subsystem12/1(In1)  "<VHAL_CAN4BusOff_flg>"
  Bus Selector1/87 -> Subsystem13/1(In1)  "<VHAL_CAN5BusOff_flg>"
  Data Type Conversion22/1 -> [VINP_CAN1BusOff_flg]  "VINP_CAN1BusOff_flg"
  Data Type Conversion23/1 -> [VINP_CAN2BusOff_flg]  "VINP_CAN2BusOff_flg"
  Data Type Conversion24/1 -> [VINP_CAN3BusOff_flg]  "VINP_CAN3BusOff_flg"
  Data Type Conversion25/1 -> [VINP_CAN4BusOff_flg]  "VINP_CAN4BusOff_flg"
  Data Type Conversion26/1 -> [VINP_CAN5BusOff_flg]  "VINP_CAN5BusOff_flg"
  [VINP_CAN1BusOff_flg] -> Bus Creator1/83
  [VINP_CAN2BusOff_flg] -> Bus Creator1/84
  [VINP_CAN3BusOff_flg] -> Bus Creator1/85
  [VINP_CAN4BusOff_flg] -> Bus Creator1/86
  [VINP_CAN5BusOff_flg] -> Bus Creator1/87
  Data Type Conversion31/1 -> [VINP_DiagRLTC_mA]  "VINP_DiagRLTC_mA"
  Data Type Conversion29/1 -> [VINP_DiagFLTC_mA]  "VINP_DiagFLTC_mA"
  Bus Selector1/95 -> Data Type Conversion32/1  "<VHAL_DiagRRTC_mA>"
  Data Type Conversion28/1 -> [VINP_DiagFMHT_s]  "VINP_DiagFMHT_s"
  Data Type Conversion32/1 -> [VINP_DiagRRTC_mA]  "VINP_DiagRRTC_mA"
  Data Type Conversion27/1 -> [VINP_DiagDRLOFF_flg]  "VINP_DiagDRLOFF_flg"
  Data Type Conversion30/1 -> [VINP_DiagFRTC_mA]  "VINP_DiagFRTC_mA"
  Bus Selector1/94 -> Data Type Conversion31/1  "<VHAL_DiagRLTC_mA>"
  Bus Selector1/92 -> Data Type Conversion29/1  "<VHAL_DiagFLTC_mA>"
  Data Type Conversion/1 -> [VINP_funAuto_flg]  "VINP_funAuto_flg"
  Bus Selector1/90 -> Data Type Conversion27/1  "<VHAL_DiagDRLOFF_flg>"
  Bus Selector1/91 -> Data Type Conversion28/1  "<VHAL_DiagFMHT_s>"
  Bus Selector1/93 -> Data Type Conversion30/1  "<VHAL_DiagFRTC_mA>"
  Bus Selector1/89 -> Data Type Conversion/1  "<VHAL_funAuto_flg>"
  Bus Selector1/96 -> Data Type Conversion33/1  "<VHAL_USSConfig_raw8>"
  Bus Selector1/97 -> Data Type Conversion34/1  "<VHAL_TireSize_raw8>"
  Bus Selector1/98 -> Data Type Conversion35/1  "<VHAL_APSFunConfig_raw8>"
  Data Type Conversion33/1 -> [VINP_USSConfig_raw8]  "VINP_USSConfig_raw8"
  Data Type Conversion34/1 -> [VINP_TireSize_raw8]  "VINP_TireSize_raw8"
  Data Type Conversion35/1 -> [VINP_APSFunConfig_raw8]  "VINP_APSFunConfig_raw8"
  Data Type Conversion36/1 -> [VINP_FlashfUnlockSingle_flg]  "VINP_FlashfUnlockSingle_flg"
  Bus Selector1/99 -> Data Type Conversion36/1  "<VHAL_FlashfUnlockSingle_flg>"
  Bus Selector1/100 -> Data Type Conversion37/1  "<VHAL_FlashRegenMode_enum>"
  Data Type Conversion37/1 -> [VINP_FlashRegenMode_enum]  "VINP_FlashRegenMode_enum"
  Data Type Conversion205/1 -> [VINP_FlashAmbBrightnessSta2_enum]  "VINP_FlashAmbBrightnessSta2_enum"
  Bus Selector1/115 -> Data Type Conversion206/1  "<VHAL_FlashAmbBrightnessSta3_enum>"
  Data Type Conversion208/1 -> [VINP_FlashAmbBrightnessSta5_enum]  "VINP_FlashAmbBrightnessSta5_enum"
  Data Type Conversion198/1 -> [VINP_FlashAmbODAEN_enum]  "VINP_FlashAmbODAEN_enum"
  Bus Selector1/105 -> Data Type Conversion197/1  "<VHAL_FlashAmbPwrWarnEN_enum>"
  Bus Selector1/103 -> Data Type Conversion195/1  "<VHAL_FlashAmbDimEN_enum>"
  Data Type Conversion203/1 -> [VINP_FlashAmbColorSta7_enum]  "VINP_FlashAmbColorSta7_enum"
  Bus Selector1/114 -> Data Type Conversion205/1  "<VHAL_FlashAmbBrightnessSta2_enum>"
  Bus Selector1/101 -> Data Type Conversion193/1  "<VHAL_FlashAmbFunEN_enum>"
  Bus Selector1/109 -> Data Type Conversion200/1  "<VHAL_FlashAmbColorSta3_enum>"
  Data Type Conversion192/1 -> [VINP_FlashAmbColorSta1_enum]  "VINP_FlashAmbColorSta1_enum"
  Data Type Conversion194/1 -> [VINP_FlashAmbWelEN_enum]  "VINP_FlashAmbWelEN_enum"
  Data Type Conversion204/1 -> [VINP_FlashAmbBrightnessSta1_enum]  "VINP_FlashAmbBrightnessSta1_enum"
  Bus Selector1/117 -> Data Type Conversion208/1  "<VHAL_FlashAmbBrightnessSta5_enum>"
  Bus Selector1/118 -> Data Type Conversion209/1  "<VHAL_FlashAmbBrightnessSta7_enum>"
  Bus Selector1/113 -> Data Type Conversion204/1  "<VHAL_FlashAmbBrightnessSta1_enum>"
  Bus Selector1/108 -> Data Type Conversion199/1  "<VHAL_FlashAmbColorSta2_enum>"
  Bus Selector1/111 -> Data Type Conversion202/1  "<VHAL_FlashAmbColorSta5_enum>"
  Bus Selector1/107 -> Data Type Conversion192/1  "<VHAL_FlashAmbColorSta1_enum>"
  Data Type Conversion209/1 -> [VINP_FlashAmbBrightnessSta7_enum]  "VINP_FlashAmbBrightnessSta7_enum"
  Bus Selector1/110 -> Data Type Conversion201/1  "<VHAL_FlashAmbColorSta4_enum>"
  Data Type Conversion196/1 -> [VINP_FlashAmbLinkDriSta_enum]  "VINP_FlashAmbLinkDriSta_enum"
  Data Type Conversion199/1 -> [VINP_FlashAmbColorSta2_enum]  "VINP_FlashAmbColorSta2_enum"
  Bus Selector1/104 -> Data Type Conversion196/1  "<VHAL_FlashAmbLinkDriSta_enum>"
  Bus Selector1/106 -> Data Type Conversion198/1  "<VHAL_FlashAmbODAEN_enum>"
  Data Type Conversion195/1 -> [VINP_FlashAmbDimEN_enum]  "VINP_FlashAmbDimEN_enum"
  Bus Selector1/112 -> Data Type Conversion203/1  "<VHAL_FlashAmbColorSta7_enum>"
  Bus Selector1/102 -> Data Type Conversion194/1  "<VHAL_FlashAmbWelEN_enum>"
  Data Type Conversion201/1 -> [VINP_FlashAmbColorSta4_enum]  "VINP_FlashAmbColorSta4_enum"
  Data Type Conversion207/1 -> [VINP_FlashAmbBrightnessSta4_enum]  "VINP_FlashAmbBrightnessSta4_enum"
  Data Type Conversion197/1 -> [VINP_FlashAmbPwrWarnEN_enum]  "VINP_FlashAmbPwrWarnEN_enum"
  Data Type Conversion206/1 -> [VINP_FlashAmbBrightnessSta3_enum]  "VINP_FlashAmbBrightnessSta3_enum"
  Data Type Conversion200/1 -> [VINP_FlashAmbColorSta3_enum]  "VINP_FlashAmbColorSta3_enum"
  Data Type Conversion202/1 -> [VINP_FlashAmbColorSta5_enum]  "VINP_FlashAmbColorSta5_enum"
  Data Type Conversion193/1 -> [VINP_FlashAmbFunEN_enum]  "VINP_FlashAmbFunEN_enum"
  Bus Selector1/116 -> Data Type Conversion207/1  "<VHAL_FlashAmbBrightnessSta4_enum>"
  Data Type Conversion39/1 -> [VINP_FlashTurnSwTSet457_enum]  "VINP_FlashTurnSwTSet457_enum"
  Bus Selector1/120 -> Data Type Conversion39/1  "<VHAL_FlashTurnSwTSet457_enum>"
  Bus Selector1/119 -> Data Type Conversion38/1  "<VHAL_FlashTurnSwTSet123_enum>"
  Data Type Conversion38/1 -> [VINP_FlashTurnSwTSet123_enum]  "VINP_FlashTurnSwTSet123_enum"
  Bus Selector1/122 -> Data Type Conversion41/1  "<VHAL_FlashREVentModeSta_enum>"
  Data Type Conversion114/1 -> [VINP_FlashLVentEN_enum]  "VINP_FlashLVentEN_enum"
  Data Type Conversion41/1 -> [VINP_FlashREVentModeSta_enum]  "VINP_FlashREVentModeSta_enum"
  Bus Selector1/129 -> Data Type Conversion47/1  "<VHAL_FlashLEVentYSta_enum>"
  Bus Selector1/126 -> Data Type Conversion45/1  "<VHAL_FlashREVentZSta_enum>"
  Bus Selector1/132 -> Data Type Conversion52/1  "<VHAL_FlashRVentEN_enum>"
  Data Type Conversion52/1 -> [VINP_FlashRVentEN_enum]  "VINP_FlashRVentEN_enum"
  Bus Selector1/135 -> Data Type Conversion50/1  "<VHAL_FlashCREVentYSta_enum>"
  Bus Selector1/121 -> Data Type Conversion40/1  "<VHAL_FlashAirIntZ3Sta_enum>"
  Bus Selector1/133 -> Data Type Conversion49/1  "<VHAL_FlashREVentYSta_enum>"
  Data Type Conversion44/1 -> [VINP_FlashCLEVentZSta_enum]  "VINP_FlashCLEVentZSta_enum"
  Bus Selector1/127 -> Data Type Conversion46/1  "<VHAL_FlashCREVentZSta_enum>"
  Bus Selector1/130 -> Data Type Conversion51/1  "<VHAL_FlashCLVentEN_enum>"
  Data Type Conversion46/1 -> [VINP_FlashCREVentZSta_enum]  "VINP_FlashCREVentZSta_enum"
  Bus Selector1/125 -> Data Type Conversion44/1  "<VHAL_FlashCLEVentZSta_enum>"
  Data Type Conversion43/1 -> [VINP_FlashLEVentZSta_enum]  "VINP_FlashLEVentZSta_enum"
  Data Type Conversion47/1 -> [VINP_FlashLEVentYSta_enum]  "VINP_FlashLEVentYSta_enum"
  Bus Selector1/134 -> Data Type Conversion115/1  "<VHAL_FlashCRVentEN_enum>"
  Data Type Conversion42/1 -> [VINP_FlashLEVentModeSta_enum]  "VINP_FlashLEVentModeSta_enum"
  Data Type Conversion51/1 -> [VINP_FlashCLVentEN_enum]  "VINP_FlashCLVentEN_enum"
  Data Type Conversion45/1 -> [VINP_FlashREVentZSta_enum]  "VINP_FlashREVentZSta_enum"
  Data Type Conversion50/1 -> [VINP_FlashCREVentYSta_enum]  "VINP_FlashCREVentYSta_enum"
  Bus Selector1/123 -> Data Type Conversion42/1  "<VHAL_FlashLEVentModeSta_enum>"
  Data Type Conversion49/1 -> [VINP_FlashREVentYSta_enum]  "VINP_FlashREVentYSta_enum"
  Bus Selector1/128 -> Data Type Conversion114/1  "<VHAL_FlashLVentEN_enum>"
  Data Type Conversion40/1 -> [VINP_FlashAirIntZ3Sta_enum]  "VINP_FlashAirIntZ3Sta_enum"
  Data Type Conversion48/1 -> [VINP_FlashCLEVentYSta_enum]  "VINP_FlashCLEVentYSta_enum"
  Bus Selector1/131 -> Data Type Conversion48/1  "<VHAL_FlashCLEVentYSta_enum>"
  Bus Selector1/124 -> Data Type Conversion43/1  "<VHAL_FlashLEVentZSta_enum>"
  Data Type Conversion115/1 -> [VINP_FlashCRVentEN_enum]  "VINP_FlashCRVentEN_enum"
  Bus Selector1/136 -> Data Type Conversion116/1  "<VHAL_FlashFGSAirIntSta_enum>"
  Bus Selector1/137 -> Data Type Conversion117/1  "<VHAL_FlashFGSChSta_enum>"
  Bus Selector1/138 -> Data Type Conversion118/1  "<VHAL_FlashFGSIONSWSta_enum>"
  Data Type Conversion116/1 -> [VINP_FlashFGSAirIntSta_enum]  "VINP_FlashFGSAirIntSta_enum"
  Data Type Conversion117/1 -> [VINP_FlashFGSChSta_enum]  "VINP_FlashFGSChSta_enum"
  Data Type Conversion118/1 -> [VINP_FlashFGSIONSWSta_enum]  "VINP_FlashFGSIONSWSta_enum"
  Data Type Conversion119/1 -> [VINP_FlashWalkOutLkEN_enum]  "VINP_FlashWalkOutLkEN_enum"
  Data Type Conversion120/1 -> [VINP_FlashWalkInUnLkEN_enum]  "VINP_FlashWalkInUnLkEN_enum"
  Data Type Conversion122/1 -> [VINP_FlashFollowMeENFun_enum]  "VINP_FlashFollowMeENFun_enum"
  Bus Selector1/139 -> Data Type Conversion119/1  "<VHAL_FlashWalkOutLkEN_enum>"
  Bus Selector1/140 -> Data Type Conversion120/1  "<VHAL_FlashWalkInUnLkEN_enum>"
  Bus Selector1/141 -> Data Type Conversion122/1  "<VHAL_FlashFollowMeENFun_enum>"
  Bus Selector1/142 -> Data Type Conversion121/1  "<VHAL_ResetPedalZeroPosReq_enum>"
  Data Type Conversion121/1 -> [VINP_ResetPedalZeroPosReq_enum]  "VINP_ResetPedalZeroPosReq_enum"
  Bus Selector1/146 -> Data Type Conversion126/1  "<VHAL_FlashPTGUserHeight4_cnt>"
  Bus Selector1/144 -> Data Type Conversion124/1  "<VHAL_FlashPTGUserHeight2_cnt>"
  Data Type Conversion127/1 -> [VINP_FlashPTGUserHeight5_cnt]  "VINP_FlashPTGUserHeight5_cnt"
  Data Type Conversion126/1 -> [VINP_FlashPTGUserHeight4_cnt]  "VINP_FlashPTGUserHeight4_cnt"
  Bus Selector1/149 -> Data Type Conversion129/1  "<VHAL_FlashPTGOpenHeight12_enum>"
  Data Type Conversion129/1 -> [VINP_FlashPTGOpenHeight12_enum]  "VINP_FlashPTGOpenHeight12_enum"
  Data Type Conversion128/1 -> [VINP_FlashPTGUserHeight7_cnt]  "VINP_FlashPTGUserHeight7_cnt"
  Bus Selector1/151 -> Data Type Conversion131/1  "<VHAL_FlashPTGOpenHeight57_enum>"
  Bus Selector1/150 -> Data Type Conversion130/1  "<VHAL_FlashPTGOpenHeight34_enum>"
  Data Type Conversion131/1 -> [VINP_FlashPTGOpenHeight57_enum]  "VINP_FlashPTGOpenHeight57_enum"
  Data Type Conversion124/1 -> [VINP_FlashPTGUserHeight2_cnt]  "VINP_FlashPTGUserHeight2_cnt"
  Bus Selector1/147 -> Data Type Conversion127/1  "<VHAL_FlashPTGUserHeight5_cnt>"
  Data Type Conversion123/1 -> [VINP_FlashPTGUserHeight1_cnt]  "VINP_FlashPTGUserHeight1_cnt"
  Bus Selector1/148 -> Data Type Conversion128/1  "<VHAL_FlashPTGUserHeight7_cnt>"
  Data Type Conversion130/1 -> [VINP_FlashPTGOpenHeight34_enum]  "VINP_FlashPTGOpenHeight34_enum"
  Data Type Conversion125/1 -> [VINP_FlashPTGUserHeight3_cnt]  "VINP_FlashPTGUserHeight3_cnt"
  Bus Selector1/143 -> Data Type Conversion123/1  "<VHAL_FlashPTGUserHeight1_cnt>"
  Bus Selector1/145 -> Data Type Conversion125/1  "<VHAL_FlashPTGUserHeight3_cnt>"
  Bus Selector1/152 -> Data Type Conversion132/1  "<VHAL_FlashACCLevelSta12_enum>"
  Bus Selector1/153 -> Data Type Conversion133/1  "<VHAL_FlashACCLevelSta34_enum>"
  Bus Selector1/154 -> Data Type Conversion134/1  "<VHAL_FlashACCLevelSta57_enum>"
  Data Type Conversion132/1 -> [VINP_FlashACCLevelSta12_enum]  "VINP_FlashACCLevelSta12_enum"
  Data Type Conversion133/1 -> [VINP_FlashACCLevelSta34_enum]  "VINP_FlashACCLevelSta34_enum"
  Data Type Conversion134/1 -> [VINP_FlashACCLevelSta57_enum]  "VINP_FlashACCLevelSta57_enum"
  Bus Selector1/155 -> Data Type Conversion137/1  "<VHAL_AutoWipHSpdEN_flg>"
  Bus Selector1/156 -> Data Type Conversion138/1  "<VHAL_WipRLSCmdHoldEN_flg>"
  Bus Selector1/157 -> Data Type Conversion135/1  "<VHAL_WipRLSCmdHoldTime_s>"
  Bus Selector1/158 -> Data Type Conversion139/1  "<VHAL_WipRLSCmdCutEN_flg>"
  Bus Selector1/159 -> Data Type Conversion136/1  "<VHAL_WipRLSCmdCutTime_s>"
  Data Type Conversion137/1 -> [VINP_AutoWipHSpdEN_flg]  "VINP_AutoWipHSpdEN_flg"
  Data Type Conversion138/1 -> [VINP_WipRLSCmdHoldEN_flg]  "VINP_WipRLSCmdHoldEN_flg"
  Data Type Conversion135/1 -> [VINP_WipRLSCmdHoldTime_s]  "VINP_WipRLSCmdHoldTime_s"
  Data Type Conversion139/1 -> [VINP_WipRLSCmdCutEN_flg]  "VINP_WipRLSCmdCutEN_flg"
  Data Type Conversion136/1 -> [VINP_WipRLSCmdCutTime_s]  "VINP_WipRLSCmdCutTime_s"
  Bus Selector1/161 -> Data Type Conversion141/1  "<VHAL_FlashAutoUnlock_enum>"
  Bus Selector1/160 -> Data Type Conversion140/1  "<VHAL_FlashAutoLock_enum>"
  Data Type Conversion141/1 -> [VINP_FlashAutoUnlock_enum]  "VINP_FlashAutoUnlock_enum"
  Data Type Conversion140/1 -> [VINP_FlashAutoLock_enum]  "VINP_FlashAutoLock_enum"
  Constant/1 -> Data Type Conversion142/1
  Data Type Conversion142/1 -> [VINP_NewNMSpec_flg]  "VINP_NewNMSpec_flg"
  Constant1/1 -> Data Type Conversion143/1
  Data Type Conversion143/1 -> [VINP_VehicleType_enum]  "VINP_VehicleType_enum"
  Constant2/1 -> Data Type Conversion144/1
  Data Type Conversion144/1 -> [VINP_SWCType_enum]  "VINP_SWCType_enum"
  Bus Selector1/162 -> Data Type Conversion145/1  "<VHAL_ECUGen1_cnt>"
  Bus Selector1/163 -> Data Type Conversion146/1  "<VHAL_ECUGen2_cnt>"
  Data Type Conversion146/1 -> [VINP_ECUGen2_cnt]  "VINP_ECUGen2_cnt"
  Data Type Conversion145/1 -> [VINP_ECUGen1_cnt]  "VINP_ECUGen1_cnt"
  Bus Selector1/88 -> Subsystem11/1(In1)  "<VHAL_CAN6BusOff_flg>"
  Data Type Conversion147/1 -> [VINP_CAN6BusOff_flg]  "VINP_CAN6BusOff_flg"
  [VINP_CAN6BusOff_flg] -> Bus Creator1/88
  [VINP_funAuto_flg] -> Bus Creator1/89
  [VINP_DiagDRLOFF_flg] -> Bus Creator1/90
  [VINP_DiagFMHT_s] -> Bus Creator1/91
  [VINP_DiagFLTC_mA] -> Bus Creator1/92
  [VINP_DiagFRTC_mA] -> Bus Creator1/93
  [VINP_DiagRLTC_mA] -> Bus Creator1/94
  [VINP_DiagRRTC_mA] -> Bus Creator1/95
  [VINP_USSConfig_raw8] -> Bus Creator1/96
  [VINP_TireSize_raw8] -> Bus Creator1/97
  [VINP_APSFunConfig_raw8] -> Bus Creator1/98
  [VINP_FlashAmbFunEN_enum] -> Bus Creator1/101
  [VINP_FlashfUnlockSingle_flg] -> Bus Creator1/99
  [VINP_FlashAmbWelEN_enum] -> Bus Creator1/102
  [VINP_FlashRegenMode_enum] -> Bus Creator1/100
  [VINP_FlashAmbDimEN_enum] -> Bus Creator1/103
  [VINP_FlashAmbLinkDriSta_enum] -> Bus Creator1/104
  [VINP_FlashAmbPwrWarnEN_enum] -> Bus Creator1/105
  [VINP_FlashAmbODAEN_enum] -> Bus Creator1/106
  [VINP_FlashAmbColorSta1_enum] -> Bus Creator1/107
  [VINP_FlashAmbColorSta2_enum] -> Bus Creator1/108
  [VINP_FlashAmbColorSta3_enum] -> Bus Creator1/109
  [VINP_FlashAmbColorSta4_enum] -> Bus Creator1/110
  [VINP_FlashAmbColorSta5_enum] -> Bus Creator1/111
  [VINP_FlashAmbColorSta7_enum] -> Bus Creator1/112
  [VINP_FlashAmbBrightnessSta1_enum] -> Bus Creator1/113
  [VINP_FlashAmbBrightnessSta2_enum] -> Bus Creator1/114
  [VINP_FlashAmbBrightnessSta3_enum] -> Bus Creator1/115
  [VINP_FlashAmbBrightnessSta4_enum] -> Bus Creator1/116
  [VINP_FlashAmbBrightnessSta5_enum] -> Bus Creator1/117
  [VINP_FlashAmbBrightnessSta7_enum] -> Bus Creator1/118
  [VINP_FlashTurnSwTSet123_enum] -> Bus Creator1/119
  [VINP_FlashTurnSwTSet457_enum] -> Bus Creator1/120
  [VINP_FlashAirIntZ3Sta_enum] -> Bus Creator1/121
  [VINP_FlashREVentModeSta_enum] -> Bus Creator1/122
  [VINP_FlashLEVentModeSta_enum] -> Bus Creator1/123
  [VINP_FlashLEVentZSta_enum] -> Bus Creator1/124
  [VINP_FlashCLEVentZSta_enum] -> Bus Creator1/125
  [VINP_FlashREVentZSta_enum] -> Bus Creator1/126
  [VINP_FlashCREVentZSta_enum] -> Bus Creator1/127
  [VINP_FlashLVentEN_enum] -> Bus Creator1/128
  [VINP_FlashLEVentYSta_enum] -> Bus Creator1/129
  [VINP_FlashCLVentEN_enum] -> Bus Creator1/130
  [VINP_FlashCLEVentYSta_enum] -> Bus Creator1/131
  [VINP_FlashRVentEN_enum] -> Bus Creator1/132
  [VINP_FlashREVentYSta_enum] -> Bus Creator1/133
  [VINP_FlashCRVentEN_enum] -> Bus Creator1/134
  [VINP_FlashCREVentYSta_enum] -> Bus Creator1/135
  [VINP_FlashFGSAirIntSta_enum] -> Bus Creator1/136
  [VINP_FlashFGSChSta_enum] -> Bus Creator1/137
  [VINP_FlashFGSIONSWSta_enum] -> Bus Creator1/138
  [VINP_FlashWalkOutLkEN_enum] -> Bus Creator1/139
  [VINP_FlashWalkInUnLkEN_enum] -> Bus Creator1/140
  [VINP_FlashFollowMeENFun_enum] -> Bus Creator1/141
  [VINP_ResetPedalZeroPosReq_enum] -> Bus Creator1/142
  [VINP_FlashPTGUserHeight1_cnt] -> Bus Creator1/143
  [VINP_FlashPTGUserHeight2_cnt] -> Bus Creator1/144
  [VINP_FlashPTGUserHeight3_cnt] -> Bus Creator1/145
  [VINP_FlashPTGUserHeight4_cnt] -> Bus Creator1/146
  [VINP_FlashPTGUserHeight5_cnt] -> Bus Creator1/147
  [VINP_FlashPTGUserHeight7_cnt] -> Bus Creator1/148
  [VINP_FlashPTGOpenHeight12_enum] -> Bus Creator1/149
  [VINP_FlashPTGOpenHeight34_enum] -> Bus Creator1/150
  [VINP_FlashPTGOpenHeight57_enum] -> Bus Creator1/151
  [VINP_NewNMSpec_flg] -> Bus Creator1/152
  [VINP_FlashACCLevelSta12_enum] -> Bus Creator1/153
  [VINP_FlashACCLevelSta34_enum] -> Bus Creator1/154
  [VINP_FlashACCLevelSta57_enum] -> Bus Creator1/155
  [VINP_AutoWipHSpdEN_flg] -> Bus Creator1/156
  [VINP_WipRLSCmdHoldEN_flg] -> Bus Creator1/157
  [VINP_WipRLSCmdHoldTime_s] -> Bus Creator1/158
  [VINP_WipRLSCmdCutEN_flg] -> Bus Creator1/159
  [VINP_WipRLSCmdCutTime_s] -> Bus Creator1/160
  [VINP_FlashAutoLock_enum] -> Bus Creator1/161
  [VINP_FlashAutoUnlock_enum] -> Bus Creator1/162
  [VINP_VehicleType_enum] -> Bus Creator1/163
  [VINP_SWCType_enum] -> Bus Creator1/164
  [VINP_ECUGen1_cnt] -> Bus Creator1/165
  [VINP_ECUGen2_cnt] -> Bus Creator1/166
  Subsystem8/1(Out1) -> Data Type Conversion22/1
  Subsystem9/1(Out1) -> Data Type Conversion23/1
  Subsystem10/1(Out1) -> Data Type Conversion24/1
  Subsystem12/1(Out1) -> Data Type Conversion25/1
  Subsystem11/1(Out1) -> Data Type Conversion147/1
  Subsystem13/1(Out1) -> Data Type Conversion26/1
  Bus Selector1/164 -> Data Type Conversion149/1  "<VHAL_FlashMILDIST_km>"
  Bus Selector1/165 -> Data Type Conversion148/1  "<VHAL_FlashWARMUPS_cnt>"
  Bus Selector1/166 -> Data Type Conversion150/1  "<VHAL_FlashCLRDIST_km>"
  Bus Selector1/167 -> Data Type Conversion151/1  "<VHAL_FlashMILTIME_min>"
  Bus Selector1/168 -> Data Type Conversion152/1  "<VHAL_FlashCLRTIME_min>"
  Bus Selector1/169 -> Data Type Conversion153/1  "<VHAL_FlashNUMPSATRIPSFLTMEMCLR_cnt>"
  Bus Selector1/170 -> Data Type Conversion154/1  "<VHAL_FlashODOMETER_km>"
  Bus Selector1/171 -> Data Type Conversion155/1  "<VHAL_FlashPSAR_sec>"
  Bus Selector1/172 -> Data Type Conversion156/1  "<VHAL_FlashPSAL_sec>"
  Bus Selector1/173 -> Data Type Conversion157/1  "<VHAL_FlashIPSAR_sec>"
  Bus Selector1/174 -> Data Type Conversion158/1  "<VHAL_FlashIPSAL_sec>"
  Bus Selector1/175 -> Data Type Conversion159/1  "<VHAL_FlashCPSAR_sec>"
  Bus Selector1/176 -> Data Type Conversion160/1  "<VHAL_FlashCPSAL_sec>"
  Bus Selector1/177 -> Data Type Conversion161/1  "<VHAL_FlashHVBNAH_Ahr>"
  Bus Selector1/178 -> Data Type Conversion162/1  "<VHAL_FlashHVBNE_kWh>"
  Bus Selector1/179 -> Data Type Conversion163/1  "<VHAL_FlashIGNCNTR_cnt>"
  Bus Selector1/180 -> Data Type Conversion164/1  "<VHAL_FlashTNBCPSAR_Ahr>"
  Bus Selector1/181 -> Data Type Conversion165/1  "<VHAL_FlashTNBCPSAL_Ahr>"
  Bus Selector1/182 -> Data Type Conversion166/1  "<VHAL_FlashTNECPSAR_kWh>"
  Bus Selector1/183 -> Data Type Conversion167/1  "<VHAL_FlashTNECPSAL_kWh>"
  Bus Selector1/184 -> Data Type Conversion168/1  "<VHAL_FlashTEBPSAR_kWh>"
  Bus Selector1/185 -> Data Type Conversion169/1  "<VHAL_FlashTEBPSAL_kWh>"
  Bus Selector1/186 -> Data Type Conversion170/1  "<VHAL_FlashTGEOVCR_kWh>"
  Bus Selector1/187 -> Data Type Conversion171/1  "<VHAL_FlashTGEOVCL_kWh>"
  Bus Selector1/188 -> Data Type Conversion172/1  "<VHAL_FlashGECHGOVCDCR_kWh>"
  Bus Selector1/189 -> Data Type Conversion173/1  "<VHAL_FlashGECHGOVCDCL_kWh>"
  Bus Selector1/190 -> Data Type Conversion174/1  "<VHAL_FlashGECHGOVCACR_kWh>"
  Bus Selector1/191 -> Data Type Conversion175/1  "<VHAL_FlashGECHGOVCACL_kWh>"
  Bus Selector1/192 -> Data Type Conversion176/1  "<VHAL_FlashRESSV2XENNONPSAR_kWh>"
  Bus Selector1/193 -> Data Type Conversion177/1  "<VHAL_FlashRESSV2XENNONPSAL_kWh>"
  Bus Selector1/194 -> Data Type Conversion178/1  "<VHAL_FlashPKERNumerator_kphsqr>"
  Bus Selector1/195 -> Data Type Conversion179/1  "<VHAL_FlashPKELNumerator_kphsqr>"
  Bus Selector1/196 -> Data Type Conversion180/1  "<VHAL_FlashResetCDEODTR_km>"
  Bus Selector1/197 -> Data Type Conversion181/1  "<VHAL_FlashAvgBattTempPSAR_C>"
  Bus Selector1/198 -> Data Type Conversion182/1  "<VHAL_FlashAvgBattTempPSAL_C>"
  Bus Selector1/199 -> Data Type Conversion183/1  "<VHAL_FlashAvgBattTempOVCR_C>"
  Bus Selector1/200 -> Data Type Conversion184/1  "<VHAL_FlashAvgBattTempOVCL_C>"
  Bus Selector1/201 -> Data Type Conversion185/1  "<VHAL_FlashAvgBattTempOFFR_C>"
  Bus Selector1/202 -> Data Type Conversion186/1  "<VHAL_FlashAvgBattTempOFFL_C>"
  Bus Selector1/203 -> Data Type Conversion187/1  "<VHAL_FlashQTYPSATRIPSR_cnt>"
  Bus Selector1/204 -> Data Type Conversion188/1  "<VHAL_FlashQTYPSATRIPSL_cnt>"
  Bus Selector1/205 -> Data Type Conversion189/1  "<VHAL_FlashRESSCNTDODRNGR_cnt>"
  Bus Selector1/206 -> Data Type Conversion190/1  "<VHAL_FlashRESSCNTDODRNGL_cnt>"
  Bus Selector1/207 -> Data Type Conversion191/1  "<VHAL_FlashETMATOER_kWh>"
  Bus Selector1/208 -> Data Type Conversion210/1  "<VHAL_FlashETMATOEL_kWh>"
  Bus Selector1/209 -> Data Type Conversion211/1  "<VHAL_FlashETMBTOER_kWh>"
  Bus Selector1/210 -> Data Type Conversion212/1  "<VHAL_FlashETMBTOEL_kWh>"
  Bus Selector1/211 -> Data Type Conversion213/1  "<VHAL_FlashRESSTIMESOCPSARNGR_s>"
  Bus Selector1/212 -> Data Type Conversion214/1  "<VHAL_FlashRESSTIMESOCPSARNGL_s>"
  Bus Selector1/213 -> Data Type Conversion215/1  "<VHAL_FlashRESSTIMESOCCHGRNGR_s>"
  Bus Selector1/214 -> Data Type Conversion216/1  "<VHAL_FlashRESSTIMESOCCHGRNGL_s>"
  Bus Selector1/215 -> Data Type Conversion217/1  "<VHAL_FlashRESSTIMESOCOFFRNGR_s>"
  Bus Selector1/216 -> Data Type Conversion218/1  "<VHAL_FlashRESSTIMESOCOFFRNGL_s>"
  Bus Selector1/217 -> Data Type Conversion219/1  "<VHAL_FlashMAXBATTEMPL_C>"
  Bus Selector1/218 -> Data Type Conversion220/1  "<VHAL_FlashMINBATTEMPL_C>"
  Bus Selector1/219 -> Data Type Conversion222/1  "<VHAL_FlashAVGBATTEMPL_sec>"
  Bus Selector1/220 -> Data Type Conversion221/1  "<VHAL_FlashAVGBATTEMPL_C>"
  Bus Selector1/221 -> Data Type Conversion223/1  "<VHAL_FlashBattTempPSAR_sec>"
  Bus Selector1/222 -> Data Type Conversion224/1  "<VHAL_FlashBattTempPSAL_sec>"
  Bus Selector1/223 -> Data Type Conversion225/1  "<VHAL_FlashOVCR_sec>"
  Bus Selector1/224 -> Data Type Conversion226/1  "<VHAL_FlashOVCL_sec>"
  Bus Selector1/225 -> Data Type Conversion227/1  "<VHAL_FlashOFFR_sec>"
  Bus Selector1/226 -> Data Type Conversion228/1  "<VHAL_FlashOFFL_sec>"
  Data Type Conversion225/1 -> [VINP_FlashOVCR_sec]  "VINP_FlashOVCR_sec"
  Data Type Conversion226/1 -> [VINP_FlashOVCL_sec]  "VINP_FlashOVCL_sec"
  Data Type Conversion162/1 -> [VINP_FlashHVBNE_kWh]  "VINP_FlashHVBNE_kWh"
  Data Type Conversion171/1 -> [VINP_FlashTGEOVCL_kWh]  "VINP_FlashTGEOVCL_kWh"
  Data Type Conversion224/1 -> [VINP_FlashBattTempPSAL_sec]  "VINP_FlashBattTempPSAL_sec"
  Data Type Conversion176/1 -> [VINP_FlashRESSV2XENNONPSAR_kWh]  "VINP_FlashRESSV2XENNONPSAR_kWh"
  Data Type Conversion175/1 -> [VINP_FlashGECHGOVCACL_kWh]  "VINP_FlashGECHGOVCACL_kWh"
  Data Type Conversion181/1 -> [VINP_FlashAvgBattTempPSAR_C]  "VINP_FlashAvgBattTempPSAR_C"
  Data Type Conversion167/1 -> [VINP_FlashTNECPSAL_kWh]  "VINP_FlashTNECPSAL_kWh"
  Data Type Conversion172/1 -> [VINP_FlashGECHGOVCDCR_kWh]  "VINP_FlashGECHGOVCDCR_kWh"
  Data Type Conversion218/1 -> [VINP_FlashRESSTIMESOCOFFRNGL_s]  "VINP_FlashRESSTIMESOCOFFRNGL_s"
  Data Type Conversion174/1 -> [VINP_FlashGECHGOVCACR_kWh]  "VINP_FlashGECHGOVCACR_kWh"
  Data Type Conversion178/1 -> [VINP_FlashPKERNumerator_kphsqr]  "VINP_FlashPKERNumerator_kphsqr"
  Data Type Conversion219/1 -> [VINP_FlashMAXBATTEMPL_C]  "VINP_FlashMAXBATTEMPL_C"
  Data Type Conversion190/1 -> [VINP_FlashRESSCNTDODRNGL_cnt]  "VINP_FlashRESSCNTDODRNGL_cnt"
  Data Type Conversion183/1 -> [VINP_FlashAvgBattTempOVCR_C]  "VINP_FlashAvgBattTempOVCR_C"
  Data Type Conversion212/1 -> [VINP_FlashETMBTOEL_kWh]  "VINP_FlashETMBTOEL_kWh"
  Data Type Conversion220/1 -> [VINP_FlashMINBATTEMPL_C]  "VINP_FlashMINBATTEMPL_C"
  Data Type Conversion223/1 -> [VINP_FlashBattTempPSAR_sec]  "VINP_FlashBattTempPSAR_sec"
  Data Type Conversion150/1 -> [VINP_FlashCLRDIST_km]  "VINP_FlashCLRDIST_km"
  Data Type Conversion214/1 -> [VINP_FlashRESSTIMESOCPSARNGL_s]  "VINP_FlashRESSTIMESOCPSARNGL_s"
  Data Type Conversion159/1 -> [VINP_FlashCPSAR_sec]  "VINP_FlashCPSAR_sec"
  Data Type Conversion173/1 -> [VINP_FlashGECHGOVCDCL_kWh]  "VINP_FlashGECHGOVCDCL_kWh"
  Data Type Conversion221/1 -> [VINP_FlashAVGBATTEMPL_C]  "VINP_FlashAVGBATTEMPL_C"
  Data Type Conversion191/1 -> [VINP_FlashETMATOER_kWh]  "VINP_FlashETMATOER_kWh"
  Data Type Conversion210/1 -> [VINP_FlashETMATOEL_kWh]  "VINP_FlashETMATOEL_kWh"
  Data Type Conversion158/1 -> [VINP_FlashIPSAL_sec]  "VINP_FlashIPSAL_sec"
  Data Type Conversion213/1 -> [VINP_FlashRESSTIMESOCPSARNGR_s]  "VINP_FlashRESSTIMESOCPSARNGR_s"
  Data Type Conversion154/1 -> [VINP_FlashODOMETER_km]  "VINP_FlashODOMETER_km"
  Data Type Conversion186/1 -> [VINP_FlashAvgBattTempOFFL_C]  "VINP_FlashAvgBattTempOFFL_C"
  Data Type Conversion228/1 -> [VINP_FlashOFFL_sec]  "VINP_FlashOFFL_sec"
  Data Type Conversion227/1 -> [VINP_FlashOFFR_sec]  "VINP_FlashOFFR_sec"
  Data Type Conversion184/1 -> [VINP_FlashAvgBattTempOVCL_C]  "VINP_FlashAvgBattTempOVCL_C"
  Data Type Conversion211/1 -> [VINP_FlashETMBTOER_kWh]  "VINP_FlashETMBTOER_kWh"
  Data Type Conversion187/1 -> [VINP_FlashQTYPSATRIPSR_cnt]  "VINP_FlashQTYPSATRIPSR_cnt"
  Data Type Conversion180/1 -> [VINP_FlashResetCDEODTR_km]  "VINP_FlashResetCDEODTR_km"
  Data Type Conversion157/1 -> [VINP_FlashIPSAR_sec]  "VINP_FlashIPSAR_sec"
  Data Type Conversion151/1 -> [VINP_FlashMILTIME_min]  "VINP_FlashMILTIME_min"
  Data Type Conversion156/1 -> [VINP_FlashPSAL_sec]  "VINP_FlashPSAL_sec"
  Data Type Conversion155/1 -> [VINP_FlashPSAR_sec]  "VINP_FlashPSAR_sec"
  Data Type Conversion169/1 -> [VINP_FlashTEBPSAL_kWh]  "VINP_FlashTEBPSAL_kWh"
  Data Type Conversion185/1 -> [VINP_FlashAvgBattTempOFFR_C]  "VINP_FlashAvgBattTempOFFR_C"
  Data Type Conversion168/1 -> [VINP_FlashTEBPSAR_kWh]  "VINP_FlashTEBPSAR_kWh"
  Data Type Conversion149/1 -> [VINP_FlashMILDIST_km]  "VINP_FlashMILDIST_km"
  Data Type Conversion217/1 -> [VINP_FlashRESSTIMESOCOFFRNGR_s]  "VINP_FlashRESSTIMESOCOFFRNGR_s"
  Data Type Conversion163/1 -> [VINP_FlashIGNCNTR_cnt]  "VINP_FlashIGNCNTR_cnt"
  Data Type Conversion179/1 -> [VINP_FlashPKELNumerator_kphsqr]  "VINP_FlashPKELNumerator_kphsqr"
  Data Type Conversion166/1 -> [VINP_FlashTNECPSAR_kWh]  "VINP_FlashTNECPSAR_kWh"
  Data Type Conversion165/1 -> [VINP_FlashTNBCPSAL_Ahr]  "VINP_FlashTNBCPSAL_Ahr"
  Data Type Conversion222/1 -> [VINP_FlashAVGBATTEMPL_sec]  "VINP_FlashAVGBATTEMPL_sec"
  Data Type Conversion153/1 -> [VINP_FlashNUMPSATRIPSFLTMEMCLR_cnt]  "VINP_FlashNUMPSATRIPSFLTMEMCLR_cnt"
  Data Type Conversion148/1 -> [VINP_FlashWARMUPS_cnt]  "VINP_FlashWARMUPS_cnt"
  Data Type Conversion170/1 -> [VINP_FlashTGEOVCR_kWh]  "VINP_FlashTGEOVCR_kWh"
  Data Type Conversion215/1 -> [VINP_FlashRESSTIMESOCCHGRNGR_s]  "VINP_FlashRESSTIMESOCCHGRNGR_s"
  Data Type Conversion188/1 -> [VINP_FlashQTYPSATRIPSL_cnt]  "VINP_FlashQTYPSATRIPSL_cnt"
  Data Type Conversion164/1 -> [VINP_FlashTNBCPSAR_Ahr]  "VINP_FlashTNBCPSAR_Ahr"
  Data Type Conversion177/1 -> [VINP_FlashRESSV2XENNONPSAL_kWh]  "VINP_FlashRESSV2XENNONPSAL_kWh"
  Data Type Conversion160/1 -> [VINP_FlashCPSAL_sec]  "VINP_FlashCPSAL_sec"
  Data Type Conversion152/1 -> [VINP_FlashCLRTIME_min]  "VINP_FlashCLRTIME_min"
  Data Type Conversion161/1 -> [VINP_FlashHVBNAH_Ahr]  "VINP_FlashHVBNAH_Ahr"
  Data Type Conversion182/1 -> [VINP_FlashAvgBattTempPSAL_C]  "VINP_FlashAvgBattTempPSAL_C"
  Data Type Conversion216/1 -> [VINP_FlashRESSTIMESOCCHGRNGL_s]  "VINP_FlashRESSTIMESOCCHGRNGL_s"
  Data Type Conversion189/1 -> [VINP_FlashRESSCNTDODRNGR_cnt]  "VINP_FlashRESSCNTDODRNGR_cnt"
  [VINP_FlashMILDIST_km] -> Bus Creator1/167
  [VINP_FlashWARMUPS_cnt] -> Bus Creator1/168
  [VINP_FlashCLRDIST_km] -> Bus Creator1/169
  [VINP_FlashMILTIME_min] -> Bus Creator1/170
  [VINP_FlashCLRTIME_min] -> Bus Creator1/171
  [VINP_FlashNUMPSATRIPSFLTMEMCLR_cnt] -> Bus Creator1/172
  [VINP_FlashODOMETER_km] -> Bus Creator1/173
  [VINP_FlashPSAR_sec] -> Bus Creator1/174
  [VINP_FlashPSAL_sec] -> Bus Creator1/175
  [VINP_FlashIPSAR_sec] -> Bus Creator1/176
  [VINP_FlashIPSAL_sec] -> Bus Creator1/177
  [VINP_FlashCPSAR_sec] -> Bus Creator1/178
  [VINP_FlashCPSAL_sec] -> Bus Creator1/179
  [VINP_FlashHVBNAH_Ahr] -> Bus Creator1/180
  [VINP_FlashHVBNE_kWh] -> Bus Creator1/181
  [VINP_FlashIGNCNTR_cnt] -> Bus Creator1/182
  [VINP_FlashTNBCPSAR_Ahr] -> Bus Creator1/183
  [VINP_FlashTNBCPSAL_Ahr] -> Bus Creator1/184
  [VINP_FlashTNECPSAR_kWh] -> Bus Creator1/185
  [VINP_FlashTNECPSAL_kWh] -> Bus Creator1/186
  [VINP_FlashTEBPSAR_kWh] -> Bus Creator1/187
  [VINP_FlashTEBPSAL_kWh] -> Bus Creator1/188
  [VINP_FlashTGEOVCR_kWh] -> Bus Creator1/189
  [VINP_FlashTGEOVCL_kWh] -> Bus Creator1/190
  [VINP_FlashGECHGOVCDCR_kWh] -> Bus Creator1/191
  [VINP_FlashGECHGOVCDCL_kWh] -> Bus Creator1/192
  [VINP_FlashGECHGOVCACR_kWh] -> Bus Creator1/193
  [VINP_FlashGECHGOVCACL_kWh] -> Bus Creator1/194
  [VINP_FlashRESSV2XENNONPSAR_kWh] -> Bus Creator1/195
  [VINP_FlashRESSV2XENNONPSAL_kWh] -> Bus Creator1/196
  [VINP_FlashPKERNumerator_kphsqr] -> Bus Creator1/197
  [VINP_FlashPKELNumerator_kphsqr] -> Bus Creator1/198
  [VINP_FlashResetCDEODTR_km] -> Bus Creator1/199
  [VINP_FlashAvgBattTempPSAR_C] -> Bus Creator1/200
  [VINP_FlashAvgBattTempPSAL_C] -> Bus Creator1/201
  [VINP_FlashAvgBattTempOVCR_C] -> Bus Creator1/202
  [VINP_FlashAvgBattTempOVCL_C] -> Bus Creator1/203
  [VINP_FlashAvgBattTempOFFR_C] -> Bus Creator1/204
  [VINP_FlashAvgBattTempOFFL_C] -> Bus Creator1/205
  [VINP_FlashQTYPSATRIPSR_cnt] -> Bus Creator1/206
  [VINP_FlashQTYPSATRIPSL_cnt] -> Bus Creator1/207
  [VINP_FlashRESSCNTDODRNGR_cnt] -> Bus Creator1/208
  [VINP_FlashRESSCNTDODRNGL_cnt] -> Bus Creator1/209
  [VINP_FlashETMATOER_kWh] -> Bus Creator1/210
  [VINP_FlashETMATOEL_kWh] -> Bus Creator1/211
  [VINP_FlashETMBTOER_kWh] -> Bus Creator1/212
  [VINP_FlashETMBTOEL_kWh] -> Bus Creator1/213
  [VINP_FlashRESSTIMESOCPSARNGR_s] -> Bus Creator1/214
  [VINP_FlashRESSTIMESOCPSARNGL_s] -> Bus Creator1/215
  [VINP_FlashRESSTIMESOCCHGRNGR_s] -> Bus Creator1/216
  [VINP_FlashRESSTIMESOCCHGRNGL_s] -> Bus Creator1/217
  [VINP_FlashRESSTIMESOCOFFRNGR_s] -> Bus Creator1/218
  [VINP_FlashRESSTIMESOCOFFRNGL_s] -> Bus Creator1/219
  [VINP_FlashMAXBATTEMPL_C] -> Bus Creator1/220
  [VINP_FlashMINBATTEMPL_C] -> Bus Creator1/221
  [VINP_FlashAVGBATTEMPL_sec] -> Bus Creator1/222
  [VINP_FlashAVGBATTEMPL_C] -> Bus Creator1/223
  [VINP_FlashBattTempPSAR_sec] -> Bus Creator1/224
  [VINP_FlashBattTempPSAL_sec] -> Bus Creator1/225
  [VINP_FlashOVCR_sec] -> Bus Creator1/226
  [VINP_FlashOVCL_sec] -> Bus Creator1/227
  [VINP_FlashOFFR_sec] -> Bus Creator1/228
  [VINP_FlashOFFL_sec] -> Bus Creator1/229
  Bus Selector1/227 -> Data Type Conversion229/1  "<VHAL_VinCode_cnt>"
  Data Type Conversion229/1 -> [VINP_VinCode_cnt]  "VINP_VinCode_cnt"
  [VINP_VinCode_cnt] -> Bus Creator1/230
  Data Type Conversion238/1 -> [VINP_FlashAutoWipHSpdEN_flg]  "VINP_FlashAutoWipHSpdEN_flg"
  Bus Selector1/232 -> Data Type Conversion234/1  "<VHAL_FlashHMIKey5Func_enum>"
  Bus Selector1/235 -> Data Type Conversion237/1  "<VHAL_FlashHMIKey8Func_enum>"
  Data Type Conversion233/1 -> [VINP_FlashHMIKey4Func_enum]  "VINP_FlashHMIKey4Func_enum"
  Bus Selector1/228 -> Data Type Conversion230/1  "<VHAL_FlashHMIKey1Func_enum>"
  Data Type Conversion231/1 -> [VINP_FlashHMIKey2Func_enum]  "VINP_FlashHMIKey2Func_enum"
  Bus Selector1/231 -> Data Type Conversion233/1  "<VHAL_FlashHMIKey4Func_enum>"
  Data Type Conversion234/1 -> [VINP_FlashHMIKey5Func_enum]  "VINP_FlashHMIKey5Func_enum"
  Data Type Conversion237/1 -> [VINP_FlashHMIKey8Func_enum]  "VINP_FlashHMIKey8Func_enum"
  Data Type Conversion236/1 -> [VINP_FlashHMIKey7Func_enum]  "VINP_FlashHMIKey7Func_enum"
  Data Type Conversion230/1 -> [VINP_FlashHMIKey1Func_enum]  "VINP_FlashHMIKey1Func_enum"
  Bus Selector1/233 -> Data Type Conversion235/1  "<VHAL_FlashHMIKey6Func_enum>"
  Bus Selector1/236 -> Data Type Conversion238/1  "<VHAL_FlashAutoWipHSpdEN_flg>"
  Bus Selector1/230 -> Data Type Conversion232/1  "<VHAL_FlashHMIKey3Func_enum>"
  Data Type Conversion232/1 -> [VINP_FlashHMIKey3Func_enum]  "VINP_FlashHMIKey3Func_enum"
  Bus Selector1/234 -> Data Type Conversion236/1  "<VHAL_FlashHMIKey7Func_enum>"
  Data Type Conversion235/1 -> [VINP_FlashHMIKey6Func_enum]  "VINP_FlashHMIKey6Func_enum"
  Bus Selector1/229 -> Data Type Conversion231/1  "<VHAL_FlashHMIKey2Func_enum>"
  [VINP_FlashHMIKey2Func_enum] -> Bus Creator1/232
  [VINP_FlashHMIKey3Func_enum] -> Bus Creator1/233
  [VINP_FlashAutoWipHSpdEN_flg] -> Bus Creator1/239
  [VINP_FlashHMIKey5Func_enum] -> Bus Creator1/235
  [VINP_FlashHMIKey6Func_enum] -> Bus Creator1/236
  [VINP_FlashHMIKey7Func_enum] -> Bus Creator1/237
  [VINP_FlashHMIKey1Func_enum] -> Bus Creator1/231
  [VINP_FlashHMIKey4Func_enum] -> Bus Creator1/234
  [VINP_FlashHMIKey8Func_enum] -> Bus Creator1/238
  Data Type Conversion240/1 -> [VINP_FlashTPMModelVersion_raw]  "VINP_FlashTPMModelVersion_raw"
  Data Type Conversion241/1 -> [VINP_FlashTPMModelVersionChkSum_raw]  "VINP_FlashTPMModelVersionChkSum_raw"
  Data Type Conversion239/1 -> [VINP_PmicBootPath_raw32]  "VINP_PmicBootPath_raw32"
  Bus Selector1/237 -> Data Type Conversion239/1  "<VHAL_PmicBootPath_raw32>"
  Bus Selector1/238 -> Data Type Conversion240/1  "<VHAL_FlashTPMModelVersion_raw>"
  Bus Selector1/239 -> Data Type Conversion241/1  "<VHAL_FlashTPMModelVersionChkSum_raw>"
  [VINP_PmicBootPath_raw32] -> Bus Creator1/240
  [VINP_FlashTPMModelVersion_raw] -> Bus Creator1/241
  [VINP_FlashTPMModelVersionChkSum_raw] -> Bus Creator1/242
  Data Type Conversion243/1 -> [VINP_FlashDIDModelVersionChkSum_raw]  "VINP_FlashDIDModelVersionChkSum_raw"
  Data Type Conversion242/1 -> [VINP_FlashDIDModelVersion_raw]  "VINP_FlashDIDModelVersion_raw"
  Bus Selector1/240 -> Data Type Conversion242/1  "<VHAL_FlashDIDModelVersion_raw>"
  Bus Selector1/241 -> Data Type Conversion243/1  "<VHAL_FlashDIDModelVersionChkSum_raw>"
  [VINP_FlashDIDModelVersion_raw] -> Bus Creator1/243
  [VINP_FlashDIDModelVersionChkSum_raw] -> Bus Creator1/244
  Data Type Conversion244/1 -> [VINP_SOCDisUsed_flg]  "VINP_SOCDisUsed_flg"
  Constant3/1 -> Data Type Conversion244/1
  [VINP_SOCDisUsed_flg] -> Bus Creator1/245
  Bus Selector1/242 -> Data Type Conversion245/1  "<VHAL_FlashAirIntenZone1MSet2_enum>"
  Bus Selector1/243 -> Data Type Conversion246/1  "<VHAL_FlashAirIntenZone1MSet3_enum>"
  Bus Selector1/244 -> Data Type Conversion247/1  "<VHAL_FlashAirIntenZone1MSet4_enum>"
  Bus Selector1/245 -> Data Type Conversion248/1  "<VHAL_FlashAirIntenZone1MSet5_enum>"
  Bus Selector1/246 -> Data Type Conversion249/1  "<VHAL_FlashAirIntenZone1MSet7_enum>"
  Bus Selector1/247 -> Data Type Conversion250/1  "<VHAL_FlashAirIntenZone3MSet2_enum>"
  Bus Selector1/248 -> Data Type Conversion251/1  "<VHAL_FlashAirIntenZone3MSet3_enum>"
  Bus Selector1/249 -> Data Type Conversion252/1  "<VHAL_FlashAirIntenZone3MSet4_enum>"
  Bus Selector1/250 -> Data Type Conversion253/1  "<VHAL_FlashAirIntenZone3MSet5_enum>"
  Bus Selector1/251 -> Data Type Conversion254/1  "<VHAL_FlashAirIntenZone3MSet7_enum>"
  Bus Selector1/252 -> Data Type Conversion255/1  "<VHAL_FlashFGSChStaSet457_enum>"
  Bus Selector1/253 -> Data Type Conversion256/1  "<VHAL_FlashFGSAirIntStaSet457_enum>"
  Bus Selector1/254 -> Data Type Conversion257/1  "<VHAL_FlashLEVentModeStaSet457_enum>"
  Bus Selector1/255 -> Data Type Conversion258/1  "<VHAL_FlashREVentModeStaSet457_enum>"
  Bus Selector1/256 -> Data Type Conversion259/1  "<VHAL_FlashLEVentZStaSet2_enum>"
  Bus Selector1/257 -> Data Type Conversion260/1  "<VHAL_FlashLEVentZStaSet3_enum>"
  Bus Selector1/258 -> Data Type Conversion261/1  "<VHAL_FlashLEVentZStaSet4_enum>"
  Bus Selector1/259 -> Data Type Conversion262/1  "<VHAL_FlashLEVentZStaSet5_enum>"
  Bus Selector1/260 -> Data Type Conversion263/1  "<VHAL_FlashLEVentZStaSet7_enum>"
  Bus Selector1/261 -> Data Type Conversion264/1  "<VHAL_FlashCLEVentZStaSet2_enum>"
  Bus Selector1/262 -> Data Type Conversion265/1  "<VHAL_FlashCLEVentZStaSet3_enum>"
  Bus Selector1/263 -> Data Type Conversion266/1  "<VHAL_FlashCLEVentZStaSet4_enum>"
  Bus Selector1/264 -> Data Type Conversion267/1  "<VHAL_FlashCLEVentZStaSet5_enum>"
  Bus Selector1/265 -> Data Type Conversion268/1  "<VHAL_FlashCLEVentZStaSet7_enum>"
  Bus Selector1/266 -> Data Type Conversion269/1  "<VHAL_FlashREVentZStaSet2_enum>"
  Bus Selector1/267 -> Data Type Conversion270/1  "<VHAL_FlashREVentZStaSet3_enum>"
  Bus Selector1/268 -> Data Type Conversion271/1  "<VHAL_FlashREVentZStaSet4_enum>"
  Bus Selector1/269 -> Data Type Conversion272/1  "<VHAL_FlashREVentZStaSet5_enum>"
  Bus Selector1/270 -> Data Type Conversion273/1  "<VHAL_FlashREVentZStaSet7_enum>"
  Bus Selector1/271 -> Data Type Conversion274/1  "<VHAL_FlashCREVentZStaSet2_enum>"
  Bus Selector1/272 -> Data Type Conversion275/1  "<VHAL_FlashCREVentZStaSet3_enum>"
  Bus Selector1/273 -> Data Type Conversion276/1  "<VHAL_FlashCREVentZStaSet4_enum>"
  Bus Selector1/274 -> Data Type Conversion277/1  "<VHAL_FlashCREVentZStaSet5_enum>"
  Bus Selector1/275 -> Data Type Conversion278/1  "<VHAL_FlashCREVentZStaSet7_enum>"
  Bus Selector1/276 -> Data Type Conversion279/1  "<VHAL_FlashLEVentYStaSet2_enum>"
  Bus Selector1/277 -> Data Type Conversion280/1  "<VHAL_FlashLEVentYStaSet3_enum>"
  Bus Selector1/278 -> Data Type Conversion281/1  "<VHAL_FlashLEVentYStaSet4_enum>"
  Bus Selector1/279 -> Data Type Conversion282/1  "<VHAL_FlashLEVentYStaSet5_enum>"
  Bus Selector1/280 -> Data Type Conversion283/1  "<VHAL_FlashLEVentYStaSet7_enum>"
  Bus Selector1/281 -> Data Type Conversion284/1  "<VHAL_FlashCLEVentYStaSet2_enum>"
  Bus Selector1/282 -> Data Type Conversion285/1  "<VHAL_FlashCLEVentYStaSet3_enum>"
  Bus Selector1/283 -> Data Type Conversion286/1  "<VHAL_FlashCLEVentYStaSet4_enum>"
  Bus Selector1/284 -> Data Type Conversion287/1  "<VHAL_FlashCLEVentYStaSet5_enum>"
  Bus Selector1/285 -> Data Type Conversion288/1  "<VHAL_FlashCLEVentYStaSet7_enum>"
  Bus Selector1/286 -> Data Type Conversion289/1  "<VHAL_FlashREVentYStaSet2_enum>"
  Bus Selector1/287 -> Data Type Conversion290/1  "<VHAL_FlashREVentYStaSet3_enum>"
  Bus Selector1/288 -> Data Type Conversion291/1  "<VHAL_FlashREVentYStaSet4_enum>"
  Bus Selector1/289 -> Data Type Conversion292/1  "<VHAL_FlashREVentYStaSet5_enum>"
  Bus Selector1/290 -> Data Type Conversion293/1  "<VHAL_FlashREVentYStaSet7_enum>"
  Bus Selector1/291 -> Data Type Conversion294/1  "<VHAL_FlashCREVentYStaSet2_enum>"
  Bus Selector1/292 -> Data Type Conversion295/1  "<VHAL_FlashCREVentYStaSet3_enum>"
  Bus Selector1/293 -> Data Type Conversion296/1  "<VHAL_FlashCREVentYStaSet4_enum>"
  Bus Selector1/294 -> Data Type Conversion297/1  "<VHAL_FlashCREVentYStaSet5_enum>"
  Bus Selector1/295 -> Data Type Conversion298/1  "<VHAL_FlashCREVentYStaSet7_enum>"
  Bus Selector1/296 -> Data Type Conversion299/1  "<VHAL_FlashACModeSet457_enum>"
  Bus Selector1/297 -> Data Type Conversion300/1  "<VHAL_FlashSettempZon1Set2_enum>"
  Bus Selector1/298 -> Data Type Conversion301/1  "<VHAL_FlashSettempZon1Set3_enum>"
  Bus Selector1/299 -> Data Type Conversion302/1  "<VHAL_FlashSettempZon1Set4_enum>"
  Bus Selector1/300 -> Data Type Conversion303/1  "<VHAL_FlashSettempZon1Set5_enum>"
  Bus Selector1/301 -> Data Type Conversion304/1  "<VHAL_FlashSettempZon1Set7_enum>"
  Data Type Conversion245/1 -> [VINP_FlashAirIntenZone1MSet2_enum]  "VINP_FlashAirIntenZone1MSet2_enum"
  Data Type Conversion246/1 -> [VINP_FlashAirIntenZone1MSet3_enum]  "VINP_FlashAirIntenZone1MSet3_enum"
  Data Type Conversion248/1 -> [VINP_FlashAirIntenZone1MSet5_enum]  "VINP_FlashAirIntenZone1MSet5_enum"
  Data Type Conversion247/1 -> [VINP_FlashAirIntenZone1MSet4_enum]  "VINP_FlashAirIntenZone1MSet4_enum"
  Data Type Conversion249/1 -> [VINP_FlashAirIntenZone1MSet7_enum]  "VINP_FlashAirIntenZone1MSet7_enum"
  Data Type Conversion250/1 -> [VINP_FlashAirIntenZone3MSet2_enum]  "VINP_FlashAirIntenZone3MSet2_enum"
  Data Type Conversion251/1 -> [VINP_FlashAirIntenZone3MSet3_enum]  "VINP_FlashAirIntenZone3MSet3_enum"
  Data Type Conversion253/1 -> [VINP_FlashAirIntenZone3MSet5_enum]  "VINP_FlashAirIntenZone3MSet5_enum"
  Data Type Conversion252/1 -> [VINP_FlashAirIntenZone3MSet4_enum]  "VINP_FlashAirIntenZone3MSet4_enum"
  Data Type Conversion254/1 -> [VINP_FlashAirIntenZone3MSet7_enum]  "VINP_FlashAirIntenZone3MSet7_enum"
  Data Type Conversion255/1 -> [VINP_FlashFGSChStaSet457_enum]  "VINP_FlashFGSChStaSet457_enum"
  Data Type Conversion256/1 -> [VINP_FlashFGSAirIntStaSet457_enum]  "VINP_FlashFGSAirIntStaSet457_enum"
  Data Type Conversion257/1 -> [VINP_FlashLEVentModeStaSet457_enum]  "VINP_FlashLEVentModeStaSet457_enum"
  Data Type Conversion258/1 -> [VINP_FlashREVentModeStaSet457_enum]  "VINP_FlashREVentModeStaSet457_enum"
  Data Type Conversion259/1 -> [VINP_FlashLEVentZStaSet2_enum]  "VINP_FlashLEVentZStaSet2_enum"
  Data Type Conversion260/1 -> [VINP_FlashLEVentZStaSet3_enum]  "VINP_FlashLEVentZStaSet3_enum"
  Data Type Conversion261/1 -> [VINP_FlashLEVentZStaSet4_enum]  "VINP_FlashLEVentZStaSet4_enum"
  Data Type Conversion263/1 -> [VINP_FlashLEVentZStaSet7_enum]  "VINP_FlashLEVentZStaSet7_enum"
  Data Type Conversion262/1 -> [VINP_FlashLEVentZStaSet5_enum]  "VINP_FlashLEVentZStaSet5_enum"
  Data Type Conversion264/1 -> [VINP_FlashCLEVentZStaSet2_enum]  "VINP_FlashCLEVentZStaSet2_enum"
  Data Type Conversion265/1 -> [VINP_FlashCLEVentZStaSet3_enum]  "VINP_FlashCLEVentZStaSet3_enum"
  Data Type Conversion266/1 -> [VINP_FlashCLEVentZStaSet4_enum]  "VINP_FlashCLEVentZStaSet4_enum"
  Data Type Conversion267/1 -> [VINP_FlashCLEVentZStaSet5_enum]  "VINP_FlashCLEVentZStaSet5_enum"
  Data Type Conversion268/1 -> [VINP_FlashCLEVentZStaSet7_enum]  "VINP_FlashCLEVentZStaSet7_enum"
  Data Type Conversion269/1 -> [VINP_FlashREVentZStaSet2_enum]  "VINP_FlashREVentZStaSet2_enum"
  Data Type Conversion270/1 -> [VINP_FlashREVentZStaSet3_enum]  "VINP_FlashREVentZStaSet3_enum"
  Data Type Conversion271/1 -> [VINP_FlashREVentZStaSet4_enum]  "VINP_FlashREVentZStaSet4_enum"
  Data Type Conversion272/1 -> [VINP_FlashREVentZStaSet5_enum]  "VINP_FlashREVentZStaSet5_enum"
  Data Type Conversion273/1 -> [VINP_FlashREVentZStaSet7_enum]  "VINP_FlashREVentZStaSet7_enum"
  Data Type Conversion274/1 -> [VINP_FlashCREVentZStaSet2_enum]  "VINP_FlashCREVentZStaSet2_enum"
  Data Type Conversion275/1 -> [VINP_FlashCREVentZStaSet3_enum]  "VINP_FlashCREVentZStaSet3_enum"
  Data Type Conversion276/1 -> [VINP_FlashCREVentZStaSet4_enum]  "VINP_FlashCREVentZStaSet4_enum"
  Data Type Conversion278/1 -> [VINP_FlashCREVentZStaSet7_enum]  "VINP_FlashCREVentZStaSet7_enum"
  Data Type Conversion277/1 -> [VINP_FlashCREVentZStaSet5_enum]  "VINP_FlashCREVentZStaSet5_enum"
  Data Type Conversion279/1 -> [VINP_FlashLEVentYStaSet2_enum]  "VINP_FlashLEVentYStaSet2_enum"
  Data Type Conversion280/1 -> [VINP_FlashLEVentYStaSet3_enum]  "VINP_FlashLEVentYStaSet3_enum"
  Data Type Conversion281/1 -> [VINP_FlashLEVentYStaSet4_enum]  "VINP_FlashLEVentYStaSet4_enum"
  Data Type Conversion283/1 -> [VINP_FlashLEVentYStaSet7_enum]  "VINP_FlashLEVentYStaSet7_enum"
  Data Type Conversion282/1 -> [VINP_FlashLEVentYStaSet5_enum]  "VINP_FlashLEVentYStaSet5_enum"
  Data Type Conversion284/1 -> [VINP_FlashCLEVentYStaSet2_enum]  "VINP_FlashCLEVentYStaSet2_enum"
  Data Type Conversion285/1 -> [VINP_FlashCLEVentYStaSet3_enum]  "VINP_FlashCLEVentYStaSet3_enum"
  Data Type Conversion286/1 -> [VINP_FlashCLEVentYStaSet4_enum]  "VINP_FlashCLEVentYStaSet4_enum"
  Data Type Conversion287/1 -> [VINP_FlashCLEVentYStaSet5_enum]  "VINP_FlashCLEVentYStaSet5_enum"
  Data Type Conversion288/1 -> [VINP_FlashCLEVentYStaSet7_enum]  "VINP_FlashCLEVentYStaSet7_enum"
  Data Type Conversion289/1 -> [VINP_FlashREVentYStaSet2_enum]  "VINP_FlashREVentYStaSet2_enum"
  Data Type Conversion290/1 -> [VINP_FlashREVentYStaSet3_enum]  "VINP_FlashREVentYStaSet3_enum"
  Data Type Conversion291/1 -> [VINP_FlashREVentYStaSet4_enum]  "VINP_FlashREVentYStaSet4_enum"
  Data Type Conversion292/1 -> [VINP_FlashREVentYStaSet5_enum]  "VINP_FlashREVentYStaSet5_enum"
  Data Type Conversion293/1 -> [VINP_FlashREVentYStaSet7_enum]  "VINP_FlashREVentYStaSet7_enum"
  Data Type Conversion294/1 -> [VINP_FlashCREVentYStaSet2_enum]  "VINP_FlashCREVentYStaSet2_enum"
  Data Type Conversion295/1 -> [VINP_FlashCREVentYStaSet3_enum]  "VINP_FlashCREVentYStaSet3_enum"
  Data Type Conversion296/1 -> [VINP_FlashCREVentYStaSet4_enum]  "VINP_FlashCREVentYStaSet4_enum"
  Data Type Conversion297/1 -> [VINP_FlashCREVentYStaSet5_enum]  "VINP_FlashCREVentYStaSet5_enum"
  Data Type Conversion298/1 -> [VINP_FlashCREVentYStaSet7_enum]  "VINP_FlashCREVentYStaSet7_enum"
  Data Type Conversion299/1 -> [VINP_FlashACModeSet457_enum]  "VINP_FlashACModeSet457_enum"
  Data Type Conversion300/1 -> [VINP_FlashSettempZon1Set2_enum]  "VINP_FlashSettempZon1Set2_enum"
  Data Type Conversion301/1 -> [VINP_FlashSettempZon1Set3_enum]  "VINP_FlashSettempZon1Set3_enum"
  Data Type Conversion302/1 -> [VINP_FlashSettempZon1Set4_enum]  "VINP_FlashSettempZon1Set4_enum"
  Data Type Conversion303/1 -> [VINP_FlashSettempZon1Set5_enum]  "VINP_FlashSettempZon1Set5_enum"
  Data Type Conversion304/1 -> [VINP_FlashSettempZon1Set7_enum]  "VINP_FlashSettempZon1Set7_enum"
  [VINP_FlashAirIntenZone1MSet2_enum] -> Bus Creator1/246
  [VINP_FlashAirIntenZone1MSet3_enum] -> Bus Creator1/247
  [VINP_FlashAirIntenZone1MSet4_enum] -> Bus Creator1/248
  [VINP_FlashAirIntenZone1MSet5_enum] -> Bus Creator1/249
  [VINP_FlashAirIntenZone1MSet7_enum] -> Bus Creator1/250
  [VINP_FlashAirIntenZone3MSet2_enum] -> Bus Creator1/251
  [VINP_FlashAirIntenZone3MSet3_enum] -> Bus Creator1/252
  [VINP_FlashAirIntenZone3MSet4_enum] -> Bus Creator1/253
  [VINP_FlashAirIntenZone3MSet5_enum] -> Bus Creator1/254
  [VINP_FlashAirIntenZone3MSet7_enum] -> Bus Creator1/255
  [VINP_FlashFGSChStaSet457_enum] -> Bus Creator1/256
  [VINP_FlashFGSAirIntStaSet457_enum] -> Bus Creator1/257
  [VINP_FlashLEVentModeStaSet457_enum] -> Bus Creator1/258
  [VINP_FlashREVentModeStaSet457_enum] -> Bus Creator1/259
  [VINP_FlashLEVentZStaSet2_enum] -> Bus Creator1/260
  [VINP_FlashLEVentZStaSet3_enum] -> Bus Creator1/261
  [VINP_FlashLEVentZStaSet4_enum] -> Bus Creator1/262
  [VINP_FlashLEVentZStaSet5_enum] -> Bus Creator1/263
  [VINP_FlashLEVentZStaSet7_enum] -> Bus Creator1/264
  [VINP_FlashCLEVentZStaSet2_enum] -> Bus Creator1/265
  [VINP_FlashCLEVentZStaSet3_enum] -> Bus Creator1/266
  [VINP_FlashCLEVentZStaSet4_enum] -> Bus Creator1/267
  [VINP_FlashCLEVentZStaSet5_enum] -> Bus Creator1/268
  [VINP_FlashCLEVentZStaSet7_enum] -> Bus Creator1/269
  [VINP_FlashREVentZStaSet2_enum] -> Bus Creator1/270
  [VINP_FlashREVentZStaSet3_enum] -> Bus Creator1/271
  [VINP_FlashREVentZStaSet4_enum] -> Bus Creator1/272
  [VINP_FlashREVentZStaSet5_enum] -> Bus Creator1/273
  [VINP_FlashREVentZStaSet7_enum] -> Bus Creator1/274
  [VINP_FlashCREVentZStaSet2_enum] -> Bus Creator1/275
  [VINP_FlashCREVentZStaSet3_enum] -> Bus Creator1/276
  [VINP_FlashCREVentZStaSet4_enum] -> Bus Creator1/277
  [VINP_FlashCREVentZStaSet5_enum] -> Bus Creator1/278
  [VINP_FlashCREVentZStaSet7_enum] -> Bus Creator1/279
  [VINP_FlashLEVentYStaSet2_enum] -> Bus Creator1/280
  [VINP_FlashLEVentYStaSet3_enum] -> Bus Creator1/281
  [VINP_FlashLEVentYStaSet4_enum] -> Bus Creator1/282
  [VINP_FlashLEVentYStaSet5_enum] -> Bus Creator1/283
  [VINP_FlashLEVentYStaSet7_enum] -> Bus Creator1/284
  [VINP_FlashCLEVentYStaSet2_enum] -> Bus Creator1/285
  [VINP_FlashCLEVentYStaSet3_enum] -> Bus Creator1/286
  [VINP_FlashCLEVentYStaSet4_enum] -> Bus Creator1/287
  [VINP_FlashCLEVentYStaSet5_enum] -> Bus Creator1/288
  [VINP_FlashCLEVentYStaSet7_enum] -> Bus Creator1/289
  [VINP_FlashREVentYStaSet2_enum] -> Bus Creator1/290
  [VINP_FlashREVentYStaSet3_enum] -> Bus Creator1/291
  [VINP_FlashREVentYStaSet4_enum] -> Bus Creator1/292
  [VINP_FlashREVentYStaSet5_enum] -> Bus Creator1/293
  [VINP_FlashREVentYStaSet7_enum] -> Bus Creator1/294
  [VINP_FlashCREVentYStaSet2_enum] -> Bus Creator1/295
  [VINP_FlashCREVentYStaSet3_enum] -> Bus Creator1/296
  [VINP_FlashCREVentYStaSet4_enum] -> Bus Creator1/297
  [VINP_FlashCREVentYStaSet5_enum] -> Bus Creator1/298
  [VINP_FlashCREVentYStaSet7_enum] -> Bus Creator1/299
  [VINP_FlashACModeSet457_enum] -> Bus Creator1/300
  [VINP_FlashSettempZon1Set2_enum] -> Bus Creator1/301
  [VINP_FlashSettempZon1Set3_enum] -> Bus Creator1/302
  [VINP_FlashSettempZon1Set4_enum] -> Bus Creator1/303
  [VINP_FlashSettempZon1Set5_enum] -> Bus Creator1/304
  [VINP_FlashSettempZon1Set7_enum] -> Bus Creator1/305
  Data Type Conversion305/1 -> [VINP_FlashJugKeepUnLZone_flg]  "VINP_FlashJugKeepUnLZone_flg"
  [VINP_FlashJugKeepUnLZone_flg] -> Bus Creator1/306
  Bus Selector1/302 -> Data Type Conversion305/1  "<VHAL_FlashJugKeepUnLZone_flg>"
  Bus Selector1/303 -> Data Type Conversion306/1  "<VHAL_DrivingMode_cnt>"
  Bus Selector1/304 -> Data Type Conversion307/1  "<VHAL_ModelYear_cnt>"
  Data Type Conversion306/1 -> [VINP_DrivingMode_cnt]  "VINP_DrivingMode_cnt"
  Data Type Conversion307/1 -> [VINP_ModelYear_cnt]  "VINP_ModelYear_cnt"
  [VINP_DrivingMode_cnt] -> Bus Creator1/307
  [VINP_ModelYear_cnt] -> Bus Creator1/308
  Bus Selector1/305 -> Data Type Conversion308/1  "<VHAL_FlashCLWinLockDrSta_enum>"
  Data Type Conversion308/1 -> [VINP_FlashCLWinLockDrSta_enum]  "VINP_FlashCLWinLockDrSta_enum"
  [VINP_FlashCLWinLockDrSta_enum] -> Bus Creator1/309
  Subsystem14/1(Out1) -> Data Type Conversion309/1
  Bus Selector1/306 -> Subsystem14/1(In1)  "<VHAL_CbnPreACEnaReq_enum>"
  Bus Selector1/307 -> Subsystem15/1(In1)  "<VHAL_PowerOffTSet_cnt>"
  Subsystem15/1(Out1) -> Data Type Conversion310/1
  Subsystem16/1(Out1) -> Data Type Conversion311/1
  Bus Selector1/308 -> Subsystem16/1(In1)  "<VHAL_ReOutsideMirror_enum>"
  Subsystem17/1(Out1) -> Data Type Conversion312/1
  Bus Selector1/309 -> Subsystem17/1(In1)  "<VHAL_ReDoorLock_enum>"
  Bus Selector1/310 -> Subsystem18/1(In1)  "<VHAL_RePwrReqTbox_enum>"
  Subsystem18/1(Out1) -> Data Type Conversion313/1
  Bus Selector1/311 -> Subsystem19/1(In1)  "<VHAL_ReRadio_flg>"
  Subsystem19/1(Out1) -> Data Type Conversion314/1
  Bus Selector1/312 -> Subsystem20/1(In1)  "<VHAL_RemoteACTemp_C>"
  Subsystem20/1(Out1) -> Data Type Conversion315/1
  Bus Selector1/313 -> Subsystem21/1(In1)  "<VHAL_RemoteAutoReq_flg>"
  Subsystem21/1(Out1) -> Data Type Conversion316/1
  Bus Selector1/314 -> Subsystem22/1(In1)  "<VHAL_TBOXRemotePW_enum>"
  Subsystem22/1(Out1) -> Data Type Conversion317/1
  Subsystem23/1(Out1) -> Data Type Conversion318/1
  Bus Selector1/315 -> Subsystem23/1(In1)  "<VHAL_FDCConnDrvWdwCtrlCmd_pct>"
  Bus Selector1/316 -> Subsystem24/1(In1)  "<VHAL_FDCConnPasWdwCtrlCmd_pct>"
  Subsystem24/1(Out1) -> Data Type Conversion319/1
  Bus Selector1/317 -> Subsystem25/1(In1)  "<VHAL_FDCConnRLDWdwCtrlCmd_pct>"
  Subsystem25/1(Out1) -> Data Type Conversion320/1
  Bus Selector1/318 -> Subsystem26/1(In1)  "<VHAL_FDCConnRRDWdwCtrlCmd_pct>"
  Subsystem26/1(Out1) -> Data Type Conversion321/1
  Data Type Conversion309/1 -> [VINP_CbnPreACEnaReq_enum]  "VINP_CbnPreACEnaReq_enum"
  Data Type Conversion310/1 -> [VINP_PowerOffTSet_cnt]  "VINP_PowerOffTSet_cnt"
  Data Type Conversion311/1 -> [VINP_ReOutsideMirror_enum]  "VINP_ReOutsideMirror_enum"
  Data Type Conversion312/1 -> [VINP_ReDoorLock_enum]  "VINP_ReDoorLock_enum"
  Data Type Conversion313/1 -> [VINP_RePwrReqTbox_enum]  "VINP_RePwrReqTbox_enum"
  Data Type Conversion314/1 -> [VINP_ReRadio_flg]  "VINP_ReRadio_flg"
  Data Type Conversion315/1 -> [VINP_RemoteACTemp_C]  "VINP_RemoteACTemp_C"
  Data Type Conversion316/1 -> [VINP_RemoteAutoReq_flg]  "VINP_RemoteAutoReq_flg"
  Data Type Conversion317/1 -> [VINP_TBOXRemotePW_enum]  "VINP_TBOXRemotePW_enum"
  Data Type Conversion318/1 -> [VINP_FDCConnDrvWdwCtrlCmd_pct]  "VINP_FDCConnDrvWdwCtrlCmd_pct"
  Data Type Conversion319/1 -> [VINP_FDCConnPasWdwCtrlCmd_pct]  "VINP_FDCConnPasWdwCtrlCmd_pct"
  Data Type Conversion320/1 -> [VINP_FDCConnRLDWdwCtrlCmd_pct]  "VINP_FDCConnRLDWdwCtrlCmd_pct"
  Data Type Conversion321/1 -> [VINP_FDCConnRRDWdwCtrlCmd_pct]  "VINP_FDCConnRRDWdwCtrlCmd_pct"
  [VINP_ReDoorLock_enum] -> Bus Creator1/313
  [VINP_ReOutsideMirror_enum] -> Bus Creator1/312
  [VINP_RePwrReqTbox_enum] -> Bus Creator1/314
  [VINP_PowerOffTSet_cnt] -> Bus Creator1/311
  [VINP_ReRadio_flg] -> Bus Creator1/315
  [VINP_RemoteACTemp_C] -> Bus Creator1/316
  [VINP_RemoteAutoReq_flg] -> Bus Creator1/317
  [VINP_CbnPreACEnaReq_enum] -> Bus Creator1/310
  [VINP_TBOXRemotePW_enum] -> Bus Creator1/318
  [VINP_FDCConnPasWdwCtrlCmd_pct] -> Bus Creator1/320
  [VINP_FDCConnRLDWdwCtrlCmd_pct] -> Bus Creator1/321
  [VINP_FDCConnDrvWdwCtrlCmd_pct] -> Bus Creator1/319
  [VINP_FDCConnRRDWdwCtrlCmd_pct] -> Bus Creator1/322
  Data Type Conversion327/1 -> [VINP_CAN6BusError_flg]  "VINP_CAN6BusError_flg"
  Data Type Conversion323/1 -> [VINP_CAN2BusError_flg]  "VINP_CAN2BusError_flg"
  Data Type Conversion324/1 -> [VINP_CAN3BusError_flg]  "VINP_CAN3BusError_flg"
  Bus Selector1/321 -> Data Type Conversion324/1  "<VHAL_CAN3BusError_flg>"
  Bus Selector1/320 -> Data Type Conversion323/1  "<VHAL_CAN2BusError_flg>"
  Bus Selector1/323 -> Data Type Conversion326/1  "<VHAL_CAN5BusError_flg>"
  Bus Selector1/324 -> Data Type Conversion327/1  "<VHAL_CAN6BusError_flg>"
  Bus Selector1/319 -> Data Type Conversion322/1  "<VHAL_CAN1BusError_flg>"
  Data Type Conversion326/1 -> [VINP_CAN5BusError_flg]  "VINP_CAN5BusError_flg"
  Data Type Conversion325/1 -> [VINP_CAN4BusError_flg]  "VINP_CAN4BusError_flg"
  Data Type Conversion322/1 -> [VINP_CAN1BusError_flg]  "VINP_CAN1BusError_flg"
  Bus Selector1/322 -> Data Type Conversion325/1  "<VHAL_CAN4BusError_flg>"
  [VINP_CAN5BusError_flg] -> Bus Creator1/327
  [VINP_CAN3BusError_flg] -> Bus Creator1/325
  [VINP_CAN4BusError_flg] -> Bus Creator1/326
  [VINP_CAN2BusError_flg] -> Bus Creator1/324
  [VINP_CAN6BusError_flg] -> Bus Creator1/328
  [VINP_CAN1BusError_flg] -> Bus Creator1/323
